simulink model "RB_dyn"  (R2024b)
settings: Solver=ode15s  StartTime=0.0  StopTime=50  RelTol=1e-4
model workspace (MAT data in the model file):
  op_trim1 = opcond.OperatingReport
  op_trim1.Outputs_(1) = opcond.OutputReport
  op_trim1.Outputs_(1).yspec_ = [-24; 8; 2.5]
  op_trim1.Outputs_(1).Block_ = 'RB_dyn/p'
  op_trim1.Outputs_(1).PortWidth_ = 3
  op_trim1.Outputs_(1).PortNumber_ = NaN
  op_trim1.Outputs_(1).y_ = [-24; 8; 2.5]
  op_trim1.Outputs_(1).Known_ = [1; 1; 1]
  op_trim1.Outputs_(1).Min_ = [-Inf; -Inf; -Inf]
  op_trim1.Outputs_(1).Max_ = [Inf; Inf; Inf]
  op_trim1.Outputs_(2) = opcond.OutputReport
  op_trim1.Outputs_(2).yspec_ = [0; 0; 0]
  op_trim1.Outputs_(2).Block_ = 'RB_dyn/omegab'
  op_trim1.Outputs_(2).PortWidth_ = 3
  op_trim1.Outputs_(2).PortNumber_ = NaN
  op_trim1.Outputs_(2).y_ = [-8.63352503319e-27; -2.14269415774e-27; 1.34149458456e-20]
  op_trim1.Outputs_(2).Known_ = [1; 1; 1]
  op_trim1.Outputs_(2).Min_ = [-Inf; -Inf; -Inf]
  op_trim1.Outputs_(2).Max_ = [Inf; Inf; Inf]
  op_trim1.Outputs_(3) = opcond.OutputReport
  op_trim1.Outputs_(3).yspec_ = [0; 0; 0]
  op_trim1.Outputs_(3).Block_ = 'RB_dyn/vi'
  op_trim1.Outputs_(3).PortWidth_ = 3
  op_trim1.Outputs_(3).PortNumber_ = NaN
  op_trim1.Outputs_(3).y_ = [7.32540041679e-34; -1.52127439379e-25; 1.31102361397e-33]
  op_trim1.Outputs_(3).Known_ = [1; 1; 1]
  op_trim1.Outputs_(3).Min_ = [-Inf; -Inf; -Inf]
  op_trim1.Outputs_(3).Max_ = [Inf; Inf; Inf]
  op_trim1.TerminationString_ = 'Operating point specifications were successfully met.'
  op_trim1.OptimizationOutput_.iterations = 4
  op_trim1.OptimizationOutput_.funcCount = 239
  op_trim1.OptimizationOutput_.lssteplength = 1
  op_trim1.OptimizationOutput_.stepsize = 3.80768589581e-07
  op_trim1.OptimizationOutput_.algorithm = 'active-set'
  op_trim1.OptimizationOutput_.firstorderopt = 9.8532065057e-08
  op_trim1.OptimizationOutput_.constrviolation = 2.27373675443e-12
  op_trim1.OptimizationOutput_.message = 'Local minimum found that satisfies the constraints.
    | 
    | Optimization completed because the objective function is non-decreasing in 
    | feasible directions, to within the value of the optimality tolerance,
    | and constraints are satisfied to within the  value of the constraint tolerance.
    | 
    | <stopping criteria details>
    | 
    | Optimization completed: The first-order optimality measure, 9.853207e-08, is less
    | than options.OptimalityTolerance = 1.000000e-06, and the maximum constraint violation,
    | 2.273737e-12,is less than options.ConstraintTolerance = 1.000000e-06.'
  op_trim1.OptimizationOutput_.bestfeasible.x = [-24; 8; 2.5; 7.32541006447e-34; -1.52127439379e-25; 1.31102361397e-33; -8.63352503319e-27; -2.14269415774e-27; 1.34149458456e-20; -24; 8; 2.5; 0; 0; 0; 6.31083339926e-17; -5.82171326753e-17; -2.42996855559e-17; -24; 8; 2.5; 819.705927891; 819.705927891; 819.705927891; 819.705927891; 819.705927891; 819.705927891; 1; -8.92792590779e-26; -9.51340523856e-35; -3.17091829691e-15; 1.43331025767e-22; 2.36799124887e-23; 8.1108698105e-17; 2.21906845952e-21; 7.27462149541e-20; 6.27728709548e-07; -1.96022275097e-15; -1.76674281195e-15; 14.715009237; -0.145; -0.145; 0; 1.39344397348e-34; -1.01153845335e-28; 6.97540031689e-29]
  op_trim1.OptimizationOutput_.bestfeasible.fval = 0
  op_trim1.OptimizationOutput_.bestfeasible.constrviolation = 2.27373675443e-12
  op_trim1.OptimizationOutput_.bestfeasible.firstorderopt = 9.8532065057e-08
  op_trim1.OptimizationOutput_.progress = {'<font face="monospaced"; size=3><BR>', 'Optimizing to solve for all desired dx/dt=0, x(k+1)-x(k)=0, and y=ydes.<BR>', ' <BR>', '(Maximum Error)  Block<BR>', ' ---------------------------------------------------------<BR>', '(1.73412e+03) RB_dyn/Allocation + Actuator Dynamics/Actuator Dynamics/Dinámica Propeller/Integrator<BR>', '(9.66614e-01) RB_dyn/Allocation + Actuator Dynamics/Actuator Dynamics/Dinámica Propeller/Integrator<BR>', '(9.52878e-01) RB_dyn/Allocation + Actuator Dynamics/Actuator Dynamics/Dinámica Propeller/Integrator<BR>', '(1.47056e-04) RB_dyn/Allocation + Actuator Dynamics/Actuator Dynamics/Dinámica Propeller/Integrator<BR>', '(2.27374e-12) RB_dyn/Allocation + Actuator Dynamics/Actuator Dynamics/Dinámica Propeller/Integrator<BR>', '(2.27374e-12) RB_dyn/Allocation + Actuator Dynamics/Actuator Dynamics/Dinámica Propeller/Integrator<BR>', ' <BR>', 'Operating point specifications were successfully met.<BR>'}
  op_trim1.Model_ = 'RB_dyn'
  op_trim1.States_(1) = opcond.StateReport
  op_trim1.States_(1).dx_ = [0; 2.27373675443e-12; 0; 0; 0; 2.27373675443e-12]
  op_trim1.States_(1).Nx_ = 6
  op_trim1.States_(1).Block_ = 'RB_dyn/Allocation + Actuator Dynamics/Actuator Dynamics/Dinámica Propeller/Integrator'
  op_trim1.States_(1).x_ = [819.705927891; 819.705927891; 819.705927891; 819.705927891; 819.705927891; 819.705927891]
  op_trim1.States_(1).SteadyState_ = [1; 1; 1; 1; 1; 1]
  op_trim1.States_(1).dxMin_ = [-Inf; -Inf; -Inf; -Inf; -Inf; -Inf]
  op_trim1.States_(1).dxMax_ = [Inf; Inf; Inf; Inf; Inf; Inf]
  op_trim1.States_(1).Known_ = [0; 0; 0; 0; 0; 0]
  op_trim1.States_(1).Min_ = [-Inf; -Inf; -Inf; -Inf; -Inf; -Inf]
  op_trim1.States_(1).Max_ = [Inf; Inf; Inf; Inf; Inf; Inf]
  op_trim1.States_(2) = opcond.StateReport
  op_trim1.States_(2).dx_ = [7.32540041679e-34; -1.52127439379e-25; 1.31102361397e-33]
  op_trim1.States_(2).Nx_ = 3
  op_trim1.States_(2).Block_ = 'RB_dyn/Dinámica UAV/Rigid Body 
    | dynamics&kinematics
    | /Velocity Integrator'
  op_trim1.States_(2).x_ = [-24; 8; 2.5]
  op_trim1.States_(2).SteadyState_ = [1; 1; 1]
  op_trim1.States_(2).dxMin_ = [-Inf; -Inf; -Inf]
  op_trim1.States_(2).dxMax_ = [Inf; Inf; Inf]
  op_trim1.States_(2).Known_ = [0; 0; 0]
  op_trim1.States_(2).Min_ = [-Inf; -Inf; -Inf]
  op_trim1.States_(2).Max_ = [Inf; Inf; Inf]
  op_trim1.States_(3) = opcond.StateReport
  op_trim1.States_(3).dx_ = [-1.86653566218e-33; 1.75165906311e-24; -1.18423789293e-15; -1.6653345369e-14; 1.11022302464e-14; 3.08218654498e-15]
  op_trim1.States_(3).Nx_ = 6
  op_trim1.States_(3).Block_ = 'RB_dyn/Dinámica UAV/Rigid Body 
    | dynamics&kinematics
    | /nu_b Integrator'
  op_trim1.States_(3).x_ = [7.32541006447e-34; -1.52127439379e-25; 1.31102361397e-33; -8.63352503319e-27; -2.14269415774e-27; 1.34149458456e-20]
  op_trim1.States_(3).SteadyState_ = [1; 1; 1; 1; 1; 1]
  op_trim1.States_(3).dxMin_ = [-Inf; -Inf; -Inf; -Inf; -Inf; -Inf]
  op_trim1.States_(3).dxMax_ = [Inf; Inf; Inf; Inf; Inf; Inf]
  op_trim1.States_(3).Known_ = [0; 0; 0; 0; 0; 0]
  op_trim1.States_(3).Min_ = [-Inf; -Inf; -Inf; -Inf; -Inf; -Inf]
  op_trim1.States_(3).Max_ = [Inf; Inf; Inf; Inf; Inf; Inf]
  op_trim1.States_(4) = opcond.StateReport
  op_trim1.States_(4).dx_ = [2.12688486169e-35; -4.31676251659e-27; -1.07134707887e-27; 6.7074729228e-21]
  op_trim1.States_(4).Nx_ = 4
  op_trim1.States_(4).Block_ = 'RB_dyn/Dinámica UAV/Rigid Body 
    | dynamics&kinematics
    | /q Integrator'
  op_trim1.States_(4).x_ = [1; -8.92792590779e-26; -9.51340523856e-35; -3.17091829691e-15]
  op_trim1.States_(4).SteadyState_ = [1; 1; 1; 1]
  op_trim1.States_(4).dxMin_ = [-Inf; -Inf; -Inf; -Inf]
  op_trim1.States_(4).dxMax_ = [Inf; Inf; Inf; Inf]
  op_trim1.States_(4).Known_ = [0; 0; 0; 0]
  op_trim1.States_(4).Min_ = [-Inf; -Inf; -Inf; -Inf]
  op_trim1.States_(4).Max_ = [Inf; Inf; Inf; Inf]
  op_trim1.States_(5) = opcond.StateReport
  op_trim1.States_(5).dx_ = [-7.32540041679e-34; 1.52127439379e-25; -1.31102361397e-33]
  op_trim1.States_(5).Nx_ = 3
  op_trim1.States_(5).Block_ = 'RB_dyn/Position Controller/ Bl Controller/ev integrator'
  op_trim1.States_(5).x_ = [1.43331025767e-22; 2.36799124887e-23; 8.1108698105e-17]
  op_trim1.States_(5).SteadyState_ = [1; 1; 1]
  op_trim1.States_(5).dxMin_ = [-Inf; -Inf; -Inf]
  op_trim1.States_(5).dxMax_ = [Inf; Inf; Inf]
  op_trim1.States_(5).Known_ = [0; 0; 0]
  op_trim1.States_(5).Min_ = [-Inf; -Inf; -Inf]
  op_trim1.States_(5).Max_ = [Inf; Inf; Inf]
  op_trim1.States_(6) = opcond.StateReport
  op_trim1.States_(6).dx_ = 1.1863912976e-33
  op_trim1.States_(6).Nx_ = 1
  op_trim1.States_(6).Block_ = 'RB_dyn/Predictor/Adaptive Laws/Projection and integration /Projection Cx/Integrator'
  op_trim1.States_(6).x_ = -1.96022275097e-15
  op_trim1.States_(6).SteadyState_ = 1
  op_trim1.States_(6).dxMin_ = -Inf
  op_trim1.States_(6).dxMax_ = Inf
  op_trim1.States_(6).Known_ = 0
  op_trim1.States_(6).Min_ = -Inf
  op_trim1.States_(6).Max_ = Inf
  op_trim1.States_(7) = opcond.StateReport
  op_trim1.States_(7).dx_ = -3.04052571068e-25
  op_trim1.States_(7).Nx_ = 1
  op_trim1.States_(7).Block_ = 'RB_dyn/Predictor/Adaptive Laws/Projection and integration /Projection Cy/Integrator'
  op_trim1.States_(7).x_ = -1.76674281195e-15
  op_trim1.States_(7).SteadyState_ = 1
  op_trim1.States_(7).dxMin_ = -Inf
  op_trim1.States_(7).dxMax_ = Inf
  op_trim1.States_(7).Known_ = 0
  op_trim1.States_(7).Min_ = -Inf
  op_trim1.States_(7).Max_ = Inf
  op_trim1.States_(8) = opcond.StateReport
  op_trim1.States_(8).dx_ = 4.65017947635e-29
  op_trim1.States_(8).Nx_ = 1
  op_trim1.States_(8).Block_ = 'RB_dyn/Predictor/Adaptive Laws/Projection and integration /Projection Cz/Integrator'
  op_trim1.States_(8).x_ = 14.715009237
  op_trim1.States_(8).SteadyState_ = 1
  op_trim1.States_(8).dxMin_ = -Inf
  op_trim1.States_(8).dxMax_ = Inf
  op_trim1.States_(8).Known_ = 0
  op_trim1.States_(8).Min_ = -Inf
  op_trim1.States_(8).Max_ = Inf
  op_trim1.States_(9) = opcond.StateReport
  op_trim1.States_(9).dx_ = 1.0489814806e-27
  op_trim1.States_(9).Nx_ = 1
  op_trim1.States_(9).Block_ = 'RB_dyn/Predictor/Adaptive Laws/Projection and integration /Projection Dx/Integrator'
  op_trim1.States_(9).x_ = -0.145
  op_trim1.States_(9).SteadyState_ = 1
  op_trim1.States_(9).dxMin_ = -Inf
  op_trim1.States_(9).dxMax_ = Inf
  op_trim1.States_(9).Known_ = 0
  op_trim1.States_(9).Min_ = -Inf
  op_trim1.States_(9).Max_ = Inf
  op_trim1.States_(10) = opcond.StateReport
  op_trim1.States_(10).dx_ = 1.0489814806e-27
  op_trim1.States_(10).Nx_ = 1
  op_trim1.States_(10).Block_ = 'RB_dyn/Predictor/Adaptive Laws/Projection and integration /Projection Dy/Integrator'
  op_trim1.States_(10).x_ = -0.145
  op_trim1.States_(10).SteadyState_ = 1
  op_trim1.States_(10).dxMin_ = -Inf
  op_trim1.States_(10).dxMax_ = Inf
  op_trim1.States_(10).Known_ = 0
  op_trim1.States_(10).Min_ = -Inf
  op_trim1.States_(10).Max_ = Inf
  op_trim1.States_(11) = opcond.StateReport
  op_trim1.States_(11).dx_ = 6.68915726758e-29
  op_trim1.States_(11).Nx_ = 1
  op_trim1.States_(11).Block_ = 'RB_dyn/Predictor/Adaptive Laws/Projection and integration /Projection Dz/Integrator'
  op_trim1.States_(11).SteadyState_ = 1
  op_trim1.States_(11).dxMin_ = -Inf
  op_trim1.States_(11).dxMax_ = Inf
  op_trim1.States_(11).Known_ = 0
  op_trim1.States_(11).Min_ = -Inf
  op_trim1.States_(11).Max_ = Inf
  op_trim1.States_(12) = opcond.StateReport
  op_trim1.States_(12).dx_ = 4.56078904608e-28
  op_trim1.States_(12).Nx_ = 1
  op_trim1.States_(12).Block_ = 'RB_dyn/Predictor/Adaptive Laws/Projection and integration /Projection lambda1/Integrator'
  op_trim1.States_(12).x_ = 2.21906845952e-21
  op_trim1.States_(12).SteadyState_ = 1
  op_trim1.States_(12).dxMin_ = -Inf
  op_trim1.States_(12).dxMax_ = Inf
  op_trim1.States_(12).Known_ = 0
  op_trim1.States_(12).Min_ = -Inf
  op_trim1.States_(12).Max_ = Inf
  op_trim1.States_(13) = opcond.StateReport
  op_trim1.States_(13).dx_ = 4.56078904608e-28
  op_trim1.States_(13).Nx_ = 1
  op_trim1.States_(13).Block_ = 'RB_dyn/Predictor/Adaptive Laws/Projection and integration /Projection lambda2/Integrator'
  op_trim1.States_(13).x_ = 7.27462149541e-20
  op_trim1.States_(13).SteadyState_ = 1
  op_trim1.States_(13).dxMin_ = -Inf
  op_trim1.States_(13).dxMax_ = Inf
  op_trim1.States_(13).Known_ = 0
  op_trim1.States_(13).Min_ = -Inf
  op_trim1.States_(13).Max_ = Inf
  op_trim1.States_(14) = opcond.StateReport
  op_trim1.States_(14).dx_ = 2.5079644533e-28
  op_trim1.States_(14).Nx_ = 1
  op_trim1.States_(14).Block_ = 'RB_dyn/Predictor/Adaptive Laws/Projection and integration /Projection lambda3/Integrator'
  op_trim1.States_(14).x_ = 6.27728709548e-07
  op_trim1.States_(14).SteadyState_ = 1
  op_trim1.States_(14).dxMin_ = -Inf
  op_trim1.States_(14).dxMax_ = Inf
  op_trim1.States_(14).Known_ = 0
  op_trim1.States_(14).Min_ = -Inf
  op_trim1.States_(14).Max_ = Inf
  op_trim1.States_(15) = opcond.StateReport
  op_trim1.States_(15).dx_ = [9.55540155376e-24; -1.12718460583e-24; -1.3950538429e-27]
  op_trim1.States_(15).Nx_ = 3
  op_trim1.States_(15).Block_ = 'RB_dyn/Predictor/Predictor Dynamics/v_hat_int'
  op_trim1.States_(15).x_ = [1.39344397348e-34; -1.01153845335e-28; 6.97540031689e-29]
  op_trim1.States_(15).SteadyState_ = [1; 1; 1]
  op_trim1.States_(15).dxMin_ = [-Inf; -Inf; -Inf]
  op_trim1.States_(15).dxMax_ = [Inf; Inf; Inf]
  op_trim1.States_(15).Known_ = [0; 0; 0]
  op_trim1.States_(15).Min_ = [-Inf; -Inf; -Inf]
  op_trim1.States_(15).Max_ = [Inf; Inf; Inf]
  op_trim1.States_(16) = opcond.StateReport
  op_trim1.States_(16).dx_ = [0; 0; 0; 0; 0; 0; 0; 0; 0]
  op_trim1.States_(16).Nx_ = 9
  op_trim1.States_(16).Block_ = 'RB_dyn/Ref State Space/Integrator'
  op_trim1.States_(16).x_ = [-24; 8; 2.5; 0; 0; 0; 6.31083339926e-17; -5.82171326753e-17; -2.42996855559e-17]
  op_trim1.States_(16).SteadyState_ = [1; 1; 1; 1; 1; 1; 1; 1; 1]
  op_trim1.States_(16).dxMin_ = [-Inf; -Inf; -Inf; -Inf; -Inf; -Inf; -Inf; -Inf; -Inf]
  op_trim1.States_(16).dxMax_ = [Inf; Inf; Inf; Inf; Inf; Inf; Inf; Inf; Inf]
  op_trim1.States_(16).Known_ = [0; 0; 0; 0; 0; 0; 0; 0; 0]
  op_trim1.States_(16).Min_ = [-Inf; -Inf; -Inf; -Inf; -Inf; -Inf; -Inf; -Inf; -Inf]
  op_trim1.States_(16).Max_ = [Inf; Inf; Inf; Inf; Inf; Inf; Inf; Inf; Inf]
  op_trim1.States_(17) = opcond.StateReport
  op_trim1.States_(17).dx_ = [0; 0; 0]
  op_trim1.States_(17).Nx_ = 3
  op_trim1.States_(17).Block_ = 'RB_dyn/V limitation/v_cmd integrator'
  op_trim1.States_(17).x_ = [-24; 8; 2.5]
  op_trim1.States_(17).SteadyState_ = [1; 1; 1]
  op_trim1.States_(17).dxMin_ = [-Inf; -Inf; -Inf]
  op_trim1.States_(17).dxMax_ = [Inf; Inf; Inf]
  op_trim1.States_(17).Known_ = [0; 0; 0]
  op_trim1.States_(17).Min_ = [-Inf; -Inf; -Inf]
  op_trim1.States_(17).Max_ = [Inf; Inf; Inf]
  op_trim2 = opcond.OperatingReport
  op_trim2.Outputs_(1) = opcond.OutputReport
  op_trim2.Outputs_(1).yspec_ = [0; 0; 0]
  op_trim2.Outputs_(1).Block_ = 'RB_dyn/p'
  op_trim2.Outputs_(1).PortWidth_ = 3
  op_trim2.Outputs_(1).PortNumber_ = NaN
  op_trim2.Outputs_(1).y_ = [0.00247480136454; 1.78220997909e-05; 1.00066556681]
  op_trim2.Outputs_(1).Known_ = [0; 0; 0]
  op_trim2.Outputs_(1).Min_ = [-Inf; -Inf; -Inf]
  op_trim2.Outputs_(1).Max_ = [Inf; Inf; Inf]
  op_trim2.Outputs_(2) = opcond.OutputReport
  op_trim2.Outputs_(2).yspec_ = [0; 0; 0]
  op_trim2.Outputs_(2).Block_ = 'RB_dyn/omegab'
  op_trim2.Outputs_(2).PortWidth_ = 3
  op_trim2.Outputs_(2).PortNumber_ = NaN
  op_trim2.Outputs_(2).y_ = [3.33045179926e-22; 5.43985403482e-20; 1.33504882827e-20]
  op_trim2.Outputs_(2).Known_ = [1; 1; 1]
  op_trim2.Outputs_(2).Min_ = [-Inf; -Inf; -Inf]
  op_trim2.Outputs_(2).Max_ = [Inf; Inf; Inf]
  op_trim2.Outputs_(3) = opcond.OutputReport
  op_trim2.Outputs_(3).yspec_ = [2; 0; 0]
  op_trim2.Outputs_(3).Block_ = 'RB_dyn/vb'
  op_trim2.Outputs_(3).PortWidth_ = 3
  op_trim2.Outputs_(3).PortNumber_ = NaN
  op_trim2.Outputs_(3).y_ = [2; 4.03619005258e-20; 4.67904532738e-20]
  op_trim2.Outputs_(3).Known_ = [1; 1; 1]
  op_trim2.Outputs_(3).Min_ = [-Inf; -Inf; -Inf]
  op_trim2.Outputs_(3).Max_ = [Inf; Inf; Inf]
  op_trim2.Outputs_(4) = opcond.OutputReport
  op_trim2.Outputs_(4).yspec_ = [0; 0; 0; 0]
  op_trim2.Outputs_(4).Block_ = 'RB_dyn/q_dot'
  op_trim2.Outputs_(4).PortWidth_ = 4
  op_trim2.Outputs_(4).PortNumber_ = NaN
  op_trim2.Outputs_(4).y_ = [-1.22708523425e-22; 2.15491260397e-22; 2.71988790305e-20; 6.67430878408e-21]
  op_trim2.Outputs_(4).Known_ = [1; 1; 1; 1]
  op_trim2.Outputs_(4).Min_ = [-Inf; -Inf; -Inf; -Inf]
  op_trim2.Outputs_(4).Max_ = [Inf; Inf; Inf; Inf]
  op_trim2.TerminationString_ = 'Operating point specifications were successfully met.'
  op_trim2.OptimizationOutput_.iterations = 4
  op_trim2.OptimizationOutput_.funcCount = 83
  op_trim2.OptimizationOutput_.lssteplength = 1
  op_trim2.OptimizationOutput_.stepsize = 0.000853707830083
  op_trim2.OptimizationOutput_.algorithm = 'active-set'
  op_trim2.OptimizationOutput_.firstorderopt = 0
  op_trim2.OptimizationOutput_.constrviolation = 4.86637581906e-09
  op_trim2.OptimizationOutput_.message = 'Local minimum found that satisfies the constraints.
    | 
    | Optimization completed because the objective function is non-decreasing in 
    | feasible directions, to within the value of the optimality tolerance,
    | and constraints are satisfied to within the  value of the constraint tolerance.
    | 
    | <stopping criteria details>
    | 
    | Optimization completed: The first-order optimality measure, 0.000000e+00, is less
    | than options.OptimalityTolerance = 1.000000e-06, and the maximum constraint violation,
    | 4.866376e-09,is less than options.ConstraintTolerance = 1.000000e-06.'
  op_trim2.OptimizationOutput_.bestfeasible.x = [0.00247480136454; 1.78220997909e-05; 1.00066556681; 2; 4.03619005258e-20; 4.67904532738e-20; 3.33045179926e-22; 5.43985403482e-20; 1.33504882827e-20; 1.00130830579; -3.05904618209e-06; 0.00467811367405; -0.000654708249021; 733.164421503; 733.163541763; 733.164247408; 733.164421503; 733.163541763; 733.164247408]
  op_trim2.OptimizationOutput_.bestfeasible.fval = 0
  op_trim2.OptimizationOutput_.bestfeasible.constrviolation = 4.86637581906e-09
  op_trim2.OptimizationOutput_.bestfeasible.firstorderopt = 0
  op_trim2.OptimizationOutput_.progress = {'<font face="monospaced"; size=3><BR>', 'Optimizing to solve for all desired dx/dt=0, x(k+1)-x(k)=0, and y=ydes.<BR>', ' <BR>', '(Maximum Error)  Block<BR>', ' ---------------------------------------------------------<BR>', '(2.00000e+00) RB_dyn/vb<BR>', '(3.56041e-04) RB_dyn/Dinámica UAV/Rigid Body  dynamics&kinematics /Integrator1<BR>', '(2.35344e-06) RB_dyn/Dinámica UAV/Rigid Body  dynamics&kinematics /Integrator1<BR>', '(4.86638e-09) RB_dyn/Dinámica UAV/Rigid Body  dynamics&kinematics /Integrator1<BR>', '(4.86638e-09) RB_dyn/Dinámica UAV/Rigid Body  dynamics&kinematics /Integrator1<BR>', ' <BR>', 'Operating point specifications were successfully met.<BR>'}
  op_trim2.Model_ = 'RB_dyn'
  op_trim2.States_(1) = opcond.StateReport
  op_trim2.States_(1).dx_ = [1.9999109815; -0.00261541012492; -0.0186875811863]
  op_trim2.States_(1).Nx_ = 3
  op_trim2.States_(1).Block_ = 'RB_dyn/Dinámica UAV/Rigid Body 
    | dynamics&kinematics
    | /Integrator'
  op_trim2.States_(1).x_ = [0.00247480136454; 1.78220997909e-05; 1.00066556681]
  op_trim2.States_(1).SteadyState_ = [0; 0; 0]
  op_trim2.States_(1).dxMin_ = [-Inf; -Inf; -Inf]
  op_trim2.States_(1).dxMax_ = [Inf; Inf; Inf]
  op_trim2.States_(1).Known_ = [0; 0; 0]
  op_trim2.States_(1).Min_ = [-Inf; -Inf; -Inf]
  op_trim2.States_(1).Max_ = [Inf; Inf; Inf]
  op_trim2.States_(2) = opcond.StateReport
  op_trim2.States_(2).dx_ = [-9.33392610888e-10; 4.86637581906e-09; 2.34032053105e-10; 9.99200562301e-14; 2.22041993795e-13; 2.31278885321e-14]
  op_trim2.States_(2).Nx_ = 6
  op_trim2.States_(2).Block_ = 'RB_dyn/Dinámica UAV/Rigid Body 
    | dynamics&kinematics
    | /Integrator1'
  op_trim2.States_(2).x_ = [2; 4.03619005258e-20; 4.67904532738e-20; 3.33045179926e-22; 5.43985403482e-20; 1.33504882827e-20]
  op_trim2.States_(2).SteadyState_ = [1; 1; 1; 1; 1; 1]
  op_trim2.States_(2).dxMin_ = [-Inf; -Inf; -Inf; -Inf; -Inf; -Inf]
  op_trim2.States_(2).dxMax_ = [Inf; Inf; Inf; Inf; Inf; Inf]
  op_trim2.States_(2).Known_ = [0; 0; 0; 0; 0; 0]
  op_trim2.States_(2).Min_ = [-Inf; -Inf; -Inf; -Inf; -Inf; -Inf]
  op_trim2.States_(2).Max_ = [Inf; Inf; Inf; Inf; Inf; Inf]
  op_trim2.States_(3) = opcond.StateReport
  op_trim2.States_(3).dx_ = [-1.22708523425e-22; 2.15491260397e-22; 2.71988790305e-20; 6.67430878408e-21]
  op_trim2.States_(3).Nx_ = 4
  op_trim2.States_(3).Block_ = 'RB_dyn/Dinámica UAV/Rigid Body 
    | dynamics&kinematics
    | /Integrator2'
  op_trim2.States_(3).x_ = [1.00130830579; -3.05904618209e-06; 0.00467811367405; -0.000654708249021]
  op_trim2.States_(3).SteadyState_ = [1; 1; 1; 1]
  op_trim2.States_(3).dxMin_ = [-Inf; -Inf; -Inf; -Inf]
  op_trim2.States_(3).dxMax_ = [Inf; Inf; Inf; Inf]
  op_trim2.States_(3).Known_ = [0; 0; 0; 0]
  op_trim2.States_(3).Min_ = [-Inf; -Inf; -Inf; -Inf]
  op_trim2.States_(3).Max_ = [Inf; Inf; Inf; Inf]
  op_trim2.Inputs_ = opcond.InputReport
  op_trim2.Inputs_.Block_ = 'RB_dyn/w_c1'
  op_trim2.Inputs_.PortWidth_ = 6
  op_trim2.Inputs_.PortDimensions_ = [2 6 1]
  op_trim2.Inputs_.u_ = [733.164421503; 733.163541763; 733.164247408; 733.164421503; 733.163541763; 733.164247408]
  op_trim2.Inputs_.Known_ = [0; 0; 0; 0; 0; 0]
  op_trim2.Inputs_.Min_ = [-Inf; -Inf; -Inf; -Inf; -Inf; -Inf]
  op_trim2.Inputs_.Max_ = [Inf; Inf; Inf; Inf; Inf; Inf]
  op_trim3 = opcond.OperatingReport
  op_trim3.Outputs_(1) = opcond.OutputReport
  op_trim3.Outputs_(1).yspec_ = [0; 0; 1]
  op_trim3.Outputs_(1).Block_ = 'RB_dyn/p'
  op_trim3.Outputs_(1).PortWidth_ = 3
  op_trim3.Outputs_(1).PortNumber_ = NaN
  op_trim3.Outputs_(1).y_ = [2; 1.8997500259e-19; 1]
  op_trim3.Outputs_(1).Known_ = [0; 1; 1]
  op_trim3.Outputs_(1).Min_ = [-Inf; -Inf; -Inf]
  op_trim3.Outputs_(1).Max_ = [Inf; Inf; Inf]
  op_trim3.Outputs_(2) = opcond.OutputReport
  op_trim3.Outputs_(2).yspec_ = [0; 0; 0]
  op_trim3.Outputs_(2).Block_ = 'RB_dyn/omegab'
  op_trim3.Outputs_(2).PortWidth_ = 3
  op_trim3.Outputs_(2).PortNumber_ = NaN
  op_trim3.Outputs_(2).y_ = [4.96522925532e-21; -1.00432731025e-20; 2.86594702329e-22]
  op_trim3.Outputs_(2).Known_ = [1; 1; 1]
  op_trim3.Outputs_(2).Min_ = [-Inf; -Inf; -Inf]
  op_trim3.Outputs_(2).Max_ = [Inf; Inf; Inf]
  op_trim3.Outputs_(3) = opcond.OutputReport
  op_trim3.Outputs_(3).yspec_ = [2; 0; 0]
  op_trim3.Outputs_(3).Block_ = 'RB_dyn/vi'
  op_trim3.Outputs_(3).PortWidth_ = 3
  op_trim3.Outputs_(3).PortNumber_ = NaN
  op_trim3.Outputs_(3).y_ = [1.99999999584; 3.36919514236e-13; 2.51599609202e-11]
  op_trim3.Outputs_(3).Known_ = [1; 1; 1]
  op_trim3.Outputs_(3).Min_ = [-Inf; -Inf; -Inf]
  op_trim3.Outputs_(3).Max_ = [Inf; Inf; Inf]
  op_trim3.Outputs_(4) = opcond.OutputReport
  op_trim3.Outputs_(4).yspec_ = [0; 0; 0; 0]
  op_trim3.Outputs_(4).Block_ = 'RB_dyn/q_dot'
  op_trim3.Outputs_(4).PortWidth_ = 4
  op_trim3.Outputs_(4).PortNumber_ = NaN
  op_trim3.Outputs_(4).y_ = [2.34608367838e-23; 2.48325700153e-21; -5.02158175194e-21; 1.31697135121e-22]
  op_trim3.Outputs_(4).Known_ = [1; 1; 1; 1]
  op_trim3.Outputs_(4).Min_ = [-Inf; -Inf; -Inf; -Inf]
  op_trim3.Outputs_(4).Max_ = [Inf; Inf; Inf; Inf]
  op_trim3.TerminationString_ = 'Operating point specifications were successfully met.'
  op_trim3.OptimizationOutput_.iterations = 3
  op_trim3.OptimizationOutput_.funcCount = 62
  op_trim3.OptimizationOutput_.lssteplength = 1
  op_trim3.OptimizationOutput_.stepsize = 2.51866712373e-07
  op_trim3.OptimizationOutput_.algorithm = 'active-set'
  op_trim3.OptimizationOutput_.firstorderopt = 0
  op_trim3.OptimizationOutput_.constrviolation = 4.16122736269e-09
  op_trim3.OptimizationOutput_.message = 'Local minimum found that satisfies the constraints.
    | 
    | Optimization completed because the objective function is non-decreasing in 
    | feasible directions, to within the value of the optimality tolerance,
    | and constraints are satisfied to within the  value of the constraint tolerance.
    | 
    | <stopping criteria details>
    | 
    | Optimization completed: The first-order optimality measure, 0.000000e+00, is less
    | than options.OptimalityTolerance = 1.000000e-06, and the maximum constraint violation,
    | 4.161227e-09,is less than options.ConstraintTolerance = 1.000000e-06.'
  op_trim3.OptimizationOutput_.bestfeasible.x = [2; 1.8997500259e-19; 1; 1.99991268736; 7.90764284672e-09; 0.0186875973027; 4.96522925532e-21; -1.00432731025e-20; 2.86594702329e-22; 0.990003847282; -9.14762811649e-12; 0.0046252992669; -1.95715128224e-09; 733.164070314; 733.164070327; 733.164070314; 733.164070314; 733.164070327; 733.164070314]
  op_trim3.OptimizationOutput_.bestfeasible.fval = 0
  op_trim3.OptimizationOutput_.bestfeasible.constrviolation = 4.16122736269e-09
  op_trim3.OptimizationOutput_.bestfeasible.firstorderopt = 0
  op_trim3.OptimizationOutput_.progress = {'<font face="monospaced"; size=3><BR>', 'Optimizing to solve for all desired dx/dt=0, x(k+1)-x(k)=0, and y=ydes.<BR>', ' <BR>', '(Maximum Error)  Block<BR>', ' ---------------------------------------------------------<BR>', '(2.00000e+00) RB_dyn/vi<BR>', '(2.27281e-02) RB_dyn/vi<BR>', '(4.16123e-09) RB_dyn/vi<BR>', '(4.16123e-09) RB_dyn/vi<BR>', ' <BR>', 'Operating point specifications were successfully met.<BR>'}
  op_trim3.Model_ = 'RB_dyn'
  op_trim3.States_(1) = opcond.StateReport
  op_trim3.States_(1).dx_ = [1.99999999584; 3.36919514236e-13; 2.51599609202e-11]
  op_trim3.States_(1).Nx_ = 3
  op_trim3.States_(1).Block_ = 'RB_dyn/Dinámica UAV/Rigid Body 
    | dynamics&kinematics
    | /Velocity Integrator'
  op_trim3.States_(1).x_ = [2; 1.8997500259e-19; 1]
  op_trim3.States_(1).SteadyState_ = [0; 1; 0]
  op_trim3.States_(1).dxMin_ = [-Inf; -Inf; -Inf]
  op_trim3.States_(1).dxMax_ = [Inf; Inf; Inf]
  op_trim3.States_(1).Known_ = [0; 0; 0]
  op_trim3.States_(1).Min_ = [-Inf; -Inf; -Inf]
  op_trim3.States_(1).Max_ = [Inf; Inf; Inf]
  op_trim3.States_(2) = opcond.StateReport
  op_trim3.States_(2).dx_ = [-7.23842280532e-14; 6.0161035039e-14; 2.75043099405e-09; -8.74300655725e-12; -3.87467787386e-12; 1.20890947797e-12]
  op_trim3.States_(2).Nx_ = 6
  op_trim3.States_(2).Block_ = 'RB_dyn/Dinámica UAV/Rigid Body 
    | dynamics&kinematics
    | /nu_b Integrator'
  op_trim3.States_(2).x_ = [1.99991268736; 7.90764284672e-09; 0.0186875973027; 4.96522925532e-21; -1.00432731025e-20; 2.86594702329e-22]
  op_trim3.States_(2).SteadyState_ = [1; 1; 1; 1; 1; 1]
  op_trim3.States_(2).dxMin_ = [-Inf; -Inf; -Inf; -Inf; -Inf; -Inf]
  op_trim3.States_(2).dxMax_ = [Inf; Inf; Inf; Inf; Inf; Inf]
  op_trim3.States_(2).Known_ = [0; 0; 0; 0; 0; 0]
  op_trim3.States_(2).Min_ = [-Inf; -Inf; -Inf; -Inf; -Inf; -Inf]
  op_trim3.States_(2).Max_ = [Inf; Inf; Inf; Inf; Inf; Inf]
  op_trim3.States_(3) = opcond.StateReport
  op_trim3.States_(3).dx_ = [2.34608367838e-23; 2.48325700153e-21; -5.02158175194e-21; 1.31697135121e-22]
  op_trim3.States_(3).Nx_ = 4
  op_trim3.States_(3).Block_ = 'RB_dyn/Dinámica UAV/Rigid Body 
    | dynamics&kinematics
    | /q Integrator'
  op_trim3.States_(3).x_ = [0.990003847282; -9.14762811649e-12; 0.0046252992669; -1.95715128224e-09]
  op_trim3.States_(3).SteadyState_ = [1; 1; 1; 1]
  op_trim3.States_(3).dxMin_ = [-Inf; -Inf; -Inf; -Inf]
  op_trim3.States_(3).dxMax_ = [Inf; Inf; Inf; Inf]
  op_trim3.States_(3).Known_ = [0; 0; 0; 0]
  op_trim3.States_(3).Min_ = [-Inf; -Inf; -Inf; -Inf]
  op_trim3.States_(3).Max_ = [Inf; Inf; Inf; Inf]
  op_trim3.Inputs_ = opcond.InputReport
  op_trim3.Inputs_.Block_ = 'RB_dyn/w_c1'
  op_trim3.Inputs_.PortWidth_ = 6
  op_trim3.Inputs_.PortDimensions_ = [2 6 1]
  op_trim3.Inputs_.u_ = [733.164070314; 733.164070327; 733.164070314; 733.164070314; 733.164070327; 733.164070314]
  op_trim3.Inputs_.Known_ = [0; 0; 0; 0; 0; 0]
  op_trim3.Inputs_.Min_ = [-Inf; -Inf; -Inf; -Inf; -Inf; -Inf]
  op_trim3.Inputs_.Max_ = [Inf; Inf; Inf; Inf; Inf; Inf]
values from neighbouring files (symbols this model uses):
  B_p = 1/(m_t_est)    [MAIN_exam_2025.m]
  F_matrix = zeros(6, 6)    [MAIN_exam_2025.m]
  Finv = pinv(F_matrix)    [MAIN_exam_2025.m]
  GAMMA_a = diag([0.5, 0.5, 0.5,1, 1, 1, 1, 1, 1, 1])    [MAIN_exam_2025.m]
  k_f = 3.65e-6    (= 3.65e-06)    [MAIN_exam_2025.m]
  K_position = diag([K_px, K_py, K_pz])    [MAIN_exam_2025.m]
  Ki = diag([K_ix, K_iy, K_iz])    [MAIN_exam_2025.m]
  Kp = diag([K_dx, K_dy, K_dz])    [MAIN_exam_2025.m]
  L = 100    [MAIN_exam_2025.m]
  LAMBDA_hat_0 = ones(3,1)    [MAIN_exam_2025.m]
  Lambda_matrix = diag([1, 1, 1, 1,1, 1])    [MAIN_exam_2025.m]
  m_t_est = UAV.m0 + m_p    [MAIN_exam_2025.m]
  omegab_0 = [0 0 0]'    [MAIN_exam_2025.m]
  p_0 = [-24 8 2.5]'    [MAIN_exam_2025.m]
  p_x_data = p_lookup(:,1)    [MAIN_exam_2025.m]
  p_y_data = p_lookup(:,2)    [MAIN_exam_2025.m]
  p_z_data = p_lookup(:,3)    [MAIN_exam_2025.m]
  q_0 = eul2quat([0, 0, 0 ]*degToRad,'XYZ')'    [MAIN_exam_2025.m]
  t_lookup = ts_pos.Time    [MAIN_exam_2025.m]
  Theta_0 = [0;0;(m_t_est)*par.g;D_fv_bar(1,1);D_fv_bar(2,2);D_fv_bar(3,3)]    [MAIN_exam_2025.m]
  v_0 = R_0*vb_0    [MAIN_exam_2025.m]
  vb_0 = [0 0 0]'    [MAIN_exam_2025.m]
undefined symbols (not defined in the file or in its folder): ctrl, par, proj, UAV
(part 1 of 2)
settings Model: PacingRate=10  Creator=justs  LastModifiedBy=fjmno
settings DataIOCC: ExternalInput=getinputstruct(op_trim1)  InitialState=getstatestruct(op_trim1)
settings OptimizationCC: ReuseModelBlockBuffer=off
settings ModelReferenceCC: EnableRefExpFcnMdlSchedulingChecks=on
settings RTWCC: GPUComputeCapability=3.5

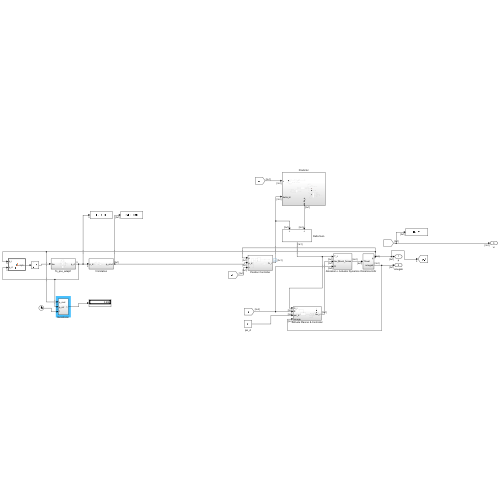
[thumbnail: Simulink's stored preview of the top-level diagram]
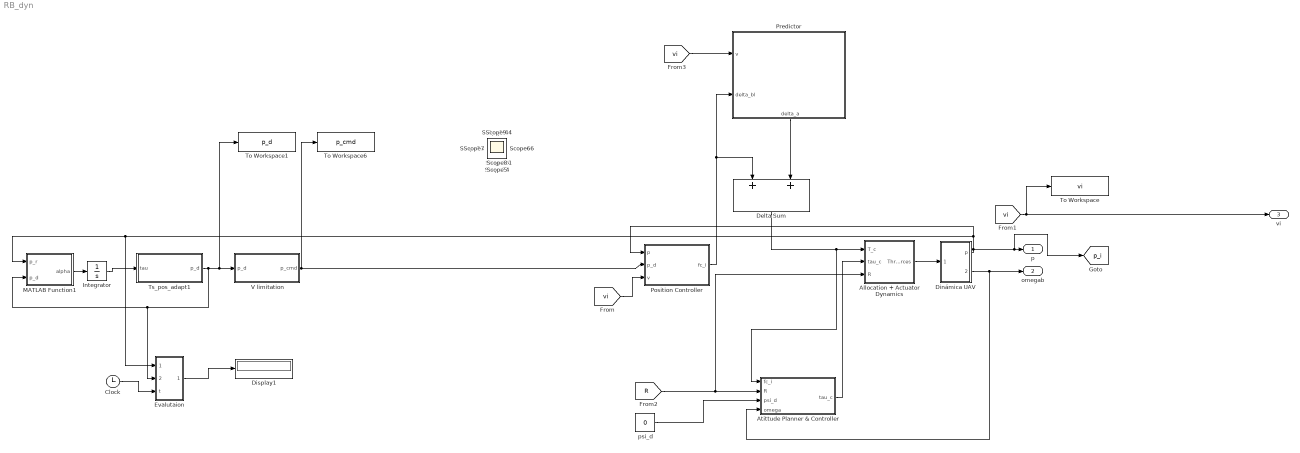
== system RB_dyn ==
  Allocation + Actuator Dynamics : Subsystem
  Atittude Planner & Controller : Subsystem
  Clock : Clock
  Delta Sum : Sum
  Dinámica UAV : Subsystem
  Display1 : Display
  Evalutaion : Subsystem
  Integrator : Integrator  LimitOutput=on  UpperSaturationLimit=100  LowerSaturationLimit=0
  MATLAB Function1 : MATLAB Function  TreatAsAtomicUnit=on
  Position Controller : Subsystem
  Predictor : Subsystem
      settings: PortSchema="{\"entries\":[{\"content\":{\"sides\":[{\"content\":{\"connectorIds\":[\"In1\",\"In2\"]},\"type\":\"ConnectorPlacement.EquallySpacedRectSide\",\"uuid\":\"2d7e5448-a673-4ee6-9554-3ae3da0510a7\"},{\"content\":{\"side\":\"RIGHT\"},\"type\":\"ConnectorPlacement.EquallySpacedRectSide\",\"uuid\":\"bdb394af-b14b-4430-b0f8-1c11ee2cd103\"},{\"content\":{\"side\":\"TOP\"},\"type\":\"ConnectorPlacement.EquallySpacedRectSide\",\"uuid\":\"33e4180b-1495-4b61-9946-a5cb762c2be0\"},{\"content\":{\"connectorIds\":[\"Out1\"],\"side\":\"BOTTOM\"},\"type\":\"ConnectorPlacement.EquallySpacedRectSide\",\"uuid\":\"431cb0aa-f168-4440-940a-a54a9a698ac8\"}]},\"type\":\"ConnectorPlacement.EquallySpacedConnector\",\"uuid\":\"3d6a6a3c-444f-43bb-b75d-620492f88baa\"}],\"packageUris\":[\"http://schema.mathworks.com/mf0/Connector/R2020b\"],\"version\":\"1.0\"}"
  To Workspace : ToWorkspace  VariableName=vi  SaveFormat=Timeseries  SampleTime=-1
  To Workspace1 : ToWorkspace  VariableName=p_d  SaveFormat=Timeseries  SampleTime=-1
  To Workspace6 : ToWorkspace  VariableName=p_cmd  SaveFormat=Timeseries  SampleTime=-1
  Ts_pos_adapt1 : Subsystem
  V limitation : Subsystem
  psi_d : Constant  Value=0
  p : Outport  PortDimensions=[3,1]
  omegab : Outport  Port=2
  vi : Outport  Port=3
  Scope{,1..14,18..21,23..24,26} (22 alike) : Scope
  tag scope: p_i=global
  wires:
  Dinámica UAV/2(omegab) -> Atittude Planner & Controller/4(omega), omegab/1
  Allocation + Actuator Dynamics/1(Thrust_forces) -> Dinámica UAV/1(Thrust)
  [R] -> Allocation + Actuator Dynamics/3(R), Atittude Planner & Controller/2(R)
  Delta Sum/1 -> Atittude Planner & Controller/1(fc_i), Allocation + Actuator Dynamics/1(T_c)
  Position Controller/1(fc_i) -> Delta Sum/1, Predictor/2(delta_bl)
  V limitation/1(p_cmd) -> Position Controller/2(p_d), To Workspace6/1
  [vi] -> Position Controller/3(v)
  [vi] -> Predictor/1(v)
  Atittude Planner & Controller/1(tau_c) -> Allocation + Actuator Dynamics/2(tau_c)
  Dinámica UAV/1(p) -> Position Controller/1(p), Evalutaion/1(p_real), MATLAB Function1/1(p_r), p/1, [p_i]
  psi_d/1 -> Atittude Planner & Controller/3(psi_d)
  MATLAB Function1/1(alpha) -> Integrator/1
  Integrator/1 -> Ts_pos_adapt1/1(tau)
  Ts_pos_adapt1/1(p_d) -> Evalutaion/2(p_ref), MATLAB Function1/2(p_d), To Workspace1/1, V limitation/1(p_d)
  Predictor/1(delta_a) -> Delta Sum/2
  Evalutaion/1(Out1) -> Display1/1
  Clock/1 -> Evalutaion/3(t)
  [vi] -> vi/1, To Workspace/1

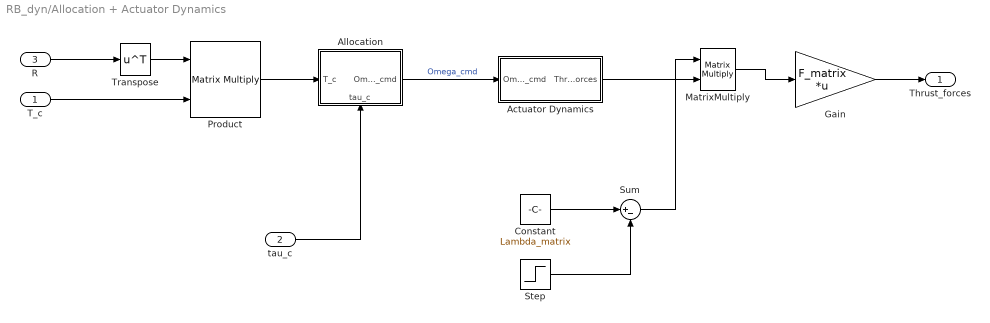
== system RB_dyn/Allocation + Actuator Dynamics ==
  T_c : Inport
  tau_c : Inport  Port=2
  R : Inport  Port=3
  Actuator Dynamics : Subsystem
  Allocation : Subsystem
      settings: PortSchema="{\"entries\":[{\"content\":{\"sides\":[{\"content\":{\"connectorIds\":[\"In1\"]},\"type\":\"ConnectorPlacement.EquallySpacedRectSide\",\"uuid\":\"27fa7930-342b-464c-b74e-3dc50cf3e81b\"},{\"content\":{\"connectorIds\":[\"Out1\"],\"side\":\"RIGHT\"},\"type\":\"ConnectorPlacement.EquallySpacedRectSide\",\"uuid\":\"52054d8e-df5f-449a-98bd-11d1376604f8\"},{\"content\":{\"side\":\"TOP\"},\"type\":\"ConnectorPlacement.EquallySpacedRectSide\",\"uuid\":\"b1419e4b-fc7c-4452-8b54-b25730e7b81d\"},{\"content\":{\"connectorIds\":[\"In2\"],\"side\":\"BOTTOM\"},\"type\":\"ConnectorPlacement.EquallySpacedRectSide\",\"uuid\":\"7ca70ec0-7c1b-4387-990e-8fb77f2b010c\"}]},\"type\":\"ConnectorPlacement.EquallySpacedConnector\",\"uuid\":\"6a86a2d4-e98f-4743-adb4-c0b70975b9c2\"}],\"packageUris\":[\"http://schema.mathworks.com/mf0/Connector/R2020b\"],\"version\":\"1.0\"}"
  Constant : Constant  Value=Lambda_matrix
  Gain : Gain  Gain=F_matrix  Multiplication=Matrix(K*u)
  MatrixMultiply : Product  Multiplication=Matrix(*)
  Product : Product  Multiplication=Matrix(*)
  Step : Step  Time=0  Before=diag([0, 0, 0, 0, 0, 0])  After=0*eye(6)  SampleTime=0
  Sum : Sum  Inputs=|+-
  Transpose : Math  Operator=transpose
  Thrust_forces : Outport
  wires:
  tau_c/1 -> Allocation/2(tau_c)
  Allocation/1(Omega_cmd) -> Actuator Dynamics/1(Omega_cmd)  "Omega_cmd"
  Product/1 -> Allocation/1(T_c)
  Transpose/1 -> Product/1
  R/1 -> Transpose/1
  T_c/1 -> Product/2
  Sum/1 -> MatrixMultiply/1
  Constant/1 -> Sum/1
  Step/1 -> Sum/2
  Gain/1 -> Thrust_forces/1
  Actuator Dynamics/1(Thrust_forces) -> MatrixMultiply/2
  MatrixMultiply/1 -> Gain/1

== system RB_dyn/Atittude Planner & Controller ==
  fc_i : Inport
  R : Inport  Port=2
  psi_d : Inport  Port=3
  omega : Inport  Port=4
  Atittude Controller : Subsystem
      settings: PortSchema="{\"entries\":[{\"content\":{\"sides\":[{\"content\":{\"connectorIds\":[\"In1\",\"In2\",\"In3\"]},\"type\":\"ConnectorPlacement.EquallySpacedRectSide\",\"uuid\":\"45854091-1ad4-48de-a2c2-5228965603de\"},{\"content\":{\"side\":\"RIGHT\"},\"type\":\"ConnectorPlacement.EquallySpacedRectSide\",\"uuid\":\"a293c214-bcaa-4f60-a42a-539eda776e35\"},{\"content\":{\"connectorIds\":[\"Out1\"],\"side\":\"TOP\"},\"type\":\"ConnectorPlacement.EquallySpacedRectSide\",\"uuid\":\"6a2ea071-b3c4-435f-ab31-1c30f1e1fcfe\"}]},\"type\":\"ConnectorPlacement.EquallySpacedConnector\",\"uuid\":\"defa2961-a4c8-4cfa-8923-ba6f5f73b83c\"}],\"packageUris\":[\"http://schema.mathworks.com/mf0/Connector/R2020b\"],\"version\":\"1.0\"}"
  Atittude Planner : Subsystem
      settings: PortSchema="{\"entries\":[{\"content\":{\"sides\":[{\"content\":{\"connectorIds\":[\"In1\"]},\"type\":\"ConnectorPlacement.EquallySpacedRectSide\",\"uuid\":\"45854091-1ad4-48de-a2c2-5228965603de\"},{\"content\":{\"connectorIds\":[\"Out1\"],\"side\":\"RIGHT\"},\"type\":\"ConnectorPlacement.EquallySpacedRectSide\",\"uuid\":\"a293c214-bcaa-4f60-a42a-539eda776e35\"},{\"content\":{\"connectorIds\":[\"In2\"],\"side\":\"TOP\"},\"type\":\"ConnectorPlacement.EquallySpacedRectSide\",\"uuid\":\"6a2ea071-b3c4-435f-ab31-1c30f1e1fcfe\"}]},\"type\":\"ConnectorPlacement.EquallySpacedConnector\",\"uuid\":\"defa2961-a4c8-4cfa-8923-ba6f5f73b83c\"}],\"packageUris\":[\"http://schema.mathworks.com/mf0/Connector/R2020b\"],\"version\":\"1.0\"}"
  tau_c : Outport
  wires:
  Atittude Planner/1(R_d) -> Atittude Controller/1(R_d)
  fc_i/1 -> Atittude Planner/2(fc_i)
  R/1 -> Atittude Controller/2(R)
  psi_d/1 -> Atittude Planner/1(psi_d)
  Atittude Controller/1(tau_c) -> tau_c/1
  omega/1 -> Atittude Controller/3(omega)

== system RB_dyn/Dinámica UAV ==
  Thrust : Inport
  Aerodynamic Damping : MATLAB Function  TreatAsAtomicUnit=on
  Gravity wrench : MATLAB Function  TreatAsAtomicUnit=on
  MATLAB Function : MATLAB Function  TreatAsAtomicUnit=on
  Matrix Divide : Product  Inputs=/*  Multiplication=Matrix(*)
  "Rigid Body dynamics&kinematics " : Subsystem
  Sum : Sum  Inputs=|+--
  p : Outport
  omegab : Outport  Port=2
  wires:
  Gravity wrench/1(w_g) -> Sum/3
  Sum/1 -> "Rigid Body dynamics&kinematics "/1(w_b)
  Aerodynamic Damping/1(D) -> Sum/2
  "Rigid Body dynamics&kinematics "/1(p) -> p/1
  "Rigid Body dynamics&kinematics "/3(vb) -> Aerodynamic Damping/1(v_b)
  "Rigid Body dynamics&kinematics "/4(omegab) -> Aerodynamic Damping/2(omega_b), omegab/1
  Thrust/1 -> Sum/1
  "Rigid Body dynamics&kinematics "/2(R) -> Matrix Divide/1, Gravity wrench/1(R)
  [p_i] -> MATLAB Function/1(p_i)
  MATLAB Function/1(vw) -> Matrix Divide/2
  Matrix Divide/1 -> Aerodynamic Damping/3(vw)

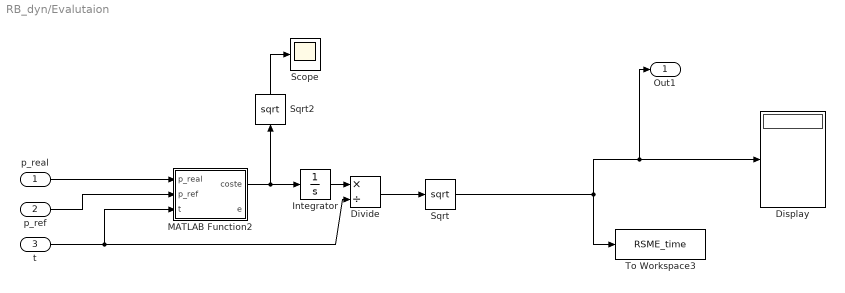
== system RB_dyn/Evalutaion ==
  p_real : Inport
  p_ref : Inport  Port=2
  t : Inport  Port=3
  Display : Display
  Divide : Product  Inputs=*/
  Integrator : Integrator
  MATLAB Function2 : MATLAB Function  TreatAsAtomicUnit=on
  Scope : Scope
  Sqrt : Sqrt  OutputSignalType=complex
  Sqrt2 : Sqrt
  To Workspace3 : ToWorkspace  VariableName=RSME_time  SaveFormat=Timeseries  SampleTime=-1
  Out1 : Outport
  wires:
  Divide/1 -> Sqrt/1
  MATLAB Function2/1(coste) -> Sqrt2/1, Integrator/1
  Sqrt/1 -> To Workspace3/1, Out1/1, Display/1
  p_ref/1 -> MATLAB Function2/2(p_ref)
  t/1 -> MATLAB Function2/3(t), Divide/2
  p_real/1 -> MATLAB Function2/1(p_real)
  Integrator/1 -> Divide/1
  Sqrt2/1 -> Scope/1

== system RB_dyn/Position Controller ==
  p : Inport
  p_d : Inport  Port=2
  v : Inport  Port=3
  " V Controller" : Subsystem
  Constant : Constant  Commented=on  Value=par.g*par.e_3
  Gain : Gain  Commented=on  Gain=m_t_est
  Pos Controller : Subsystem
      settings: PortSchema="{\"entries\":[{\"content\":{\"sides\":[{\"content\":{},\"type\":\"ConnectorPlacement.EquallySpacedRectSide\",\"uuid\":\"2fb879fa-9caa-4b67-ad1c-6d77d0280c38\"},{\"content\":{\"connectorIds\":[\"Out1\"],\"side\":\"RIGHT\"},\"type\":\"ConnectorPlacement.EquallySpacedRectSide\",\"uuid\":\"82fa2ff9-e48a-4751-98bb-12047787667e\"},{\"content\":{\"side\":\"TOP\"},\"type\":\"ConnectorPlacement.EquallySpacedRectSide\",\"uuid\":\"70e781bb-fb0f-473c-82a2-e9ed483c0d65\"},{\"content\":{\"connectorIds\":[\"In1\",\"In2\"],\"side\":\"BOTTOM\"},\"type\":\"ConnectorPlacement.EquallySpacedRectSide\",\"uuid\":\"1bc1f217-6b4c-4a6c-b3cf-0622d8ade2ed\"}]},\"type\":\"ConnectorPlacement.EquallySpacedConnector\",\"uuid\":\"d006ffe8-6230-4662-ba3a-e7870a3b1b43\"}],\"packageUris\":[\"http://schema.mathworks.com/mf0/Connector/R2020b\"],\"version\":\"1.0\"}"
  Sum : Sum  Inputs=|++
  fc_i : Outport
  wires:
  p_d/1 -> Pos Controller/1(p_cmd)
  Pos Controller/1(v_cmd) -> " V Controller"/1(v_cmd)
  v/1 -> " V Controller"/2(v)
  p/1 -> Pos Controller/2(p)
  " V Controller"/1(u_bl) -> Sum/1
  Constant/1 -> Gain/1
  Gain/1 -> Sum/2
  Sum/1 -> fc_i/1

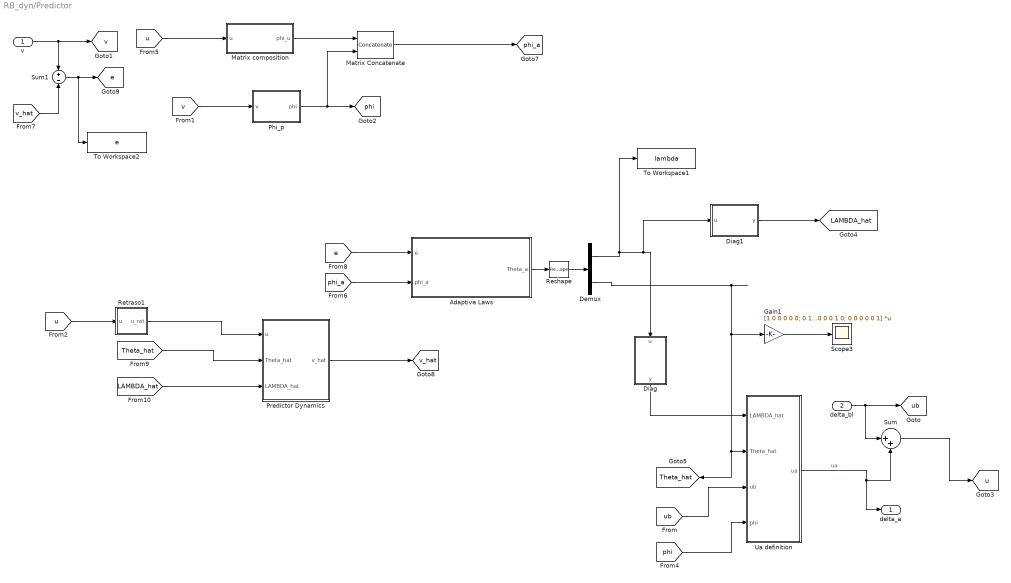
== system RB_dyn/Predictor ==
  v : Inport
  delta_bl : Inport  Port=2
  Adaptive Laws : Subsystem
  Demux : Demux  Outputs=[3,6]
  Diag : MATLAB Function  TreatAsAtomicUnit=on
  Diag1 : MATLAB Function  TreatAsAtomicUnit=on
  Gain1 : Gain  Gain=[1 0 0 0 0 0; 0 1 0 0 0 0;0 0 0 1 0 0; 0 0 0 0 1 0; 0 0 0 0 0 1]  Multiplication=Matrix(K*u)
  Matrix Concatenate : Concatenate  Mode=Multidimensional array
  Matrix composition : Subsystem
  Phi_p : MATLAB Function  TreatAsAtomicUnit=on
  Predictor Dynamics : Subsystem
  Reshape : Reshape  OutputDimensionality=Column vector (2-D)
  Retraso1 : Subsystem
  Scope3 : Scope
  Sum : Sum  Inputs=|++
  Sum1 : Sum  Inputs=+-
  To Workspace1 : ToWorkspace  VariableName=lambda  SaveFormat=Timeseries  SampleTime=-1
  To Workspace2 : ToWorkspace  VariableName=e  SaveFormat=Timeseries  SampleTime=-1
  Ua definition : Subsystem
  delta_a : Outport  PortDimensions=[3,1]
  tag scope: LAMBDA_hat=global, Theta_hat=global, e=global, phi=global, phi_a=global, u=global, ub=global, v=global, v_hat=global
  wires:
  Ua definition/1(ua) -> delta_a/1, Sum/2  "ua"
  Sum/1 -> [u]
  delta_bl/1 -> [ub], Sum/1
  v/1 -> Sum1/1, [v]
  [ub] -> Ua definition/3(ub)
  [v] -> Phi_p/1(v)
  Phi_p/1(phi) -> Matrix Concatenate/2, [phi]
  [u] -> Retraso1/1(u)
  [phi] -> Ua definition/4(phi)
  Adaptive Laws/1(Theta_a) -> Reshape/1
  Demux/1 -> Diag/1(u), Diag1/1(u), To Workspace1/1
  Matrix Concatenate/1 -> [phi_a]
  [phi_a] -> Adaptive Laws/2(phi_a)
  Predictor Dynamics/1(v_hat) -> [v_hat]
  [v_hat] -> Sum1/2
  Sum1/1 -> To Workspace2/1, [e]
  [e] -> Adaptive Laws/1(e)
  [Theta_hat] -> Predictor Dynamics/2(Theta_hat)
  [LAMBDA_hat] -> Predictor Dynamics/3(LAMBDA_hat)
  Demux/2 -> Gain1/1, [Theta_hat], Ua definition/2(Theta_hat)
  Matrix composition/1(phi_u) -> Matrix Concatenate/1
  Diag/1(y) -> Ua definition/1(LAMBDA_hat)
  Reshape/1 -> Demux/1
  Diag1/1(y) -> [LAMBDA_hat]
  Retraso1/1(u_ret) -> Predictor Dynamics/1(u)
  [u] -> Matrix composition/1(u)
  Gain1/1 -> Scope3/1

== system RB_dyn/Ts_pos_adapt1 ==
  tau : Inport
  1-D Lookup Table : Lookup_n-D  NumberOfTableDimensions=1  BreakpointsForDimension1=t_lookup  Table=p_x_data  ExtrapMethod=Clip  InternalRulePriority=Speed  RndMeth=Simplest
  1-D Lookup Table1 : Lookup_n-D  NumberOfTableDimensions=1  BreakpointsForDimension1=t_lookup  Table=p_y_data  ExtrapMethod=Clip  InternalRulePriority=Speed  RndMeth=Simplest
  1-D Lookup Table2 : Lookup_n-D  NumberOfTableDimensions=1  BreakpointsForDimension1=t_lookup  Table=p_z_data  ExtrapMethod=Clip  InternalRulePriority=Speed  RndMeth=Simplest
  Mux : Mux  Inputs=3
  p_d : Outport
  wires:
  tau/1 -> 1-D Lookup Table1/1, 1-D Lookup Table/1, 1-D Lookup Table2/1
  1-D Lookup Table/1 -> Mux/1
  1-D Lookup Table1/1 -> Mux/2
  1-D Lookup Table2/1 -> Mux/3
  Mux/1 -> p_d/1

== system RB_dyn/V limitation ==
  p_d : Inport
  Gain : Gain  Gain=K_position  Multiplication=Matrix(K*u)
  Scope : Scope
  Scope1 : Scope
  Sum : Sum  Inputs=+-
  V_limitation : MATLAB Function  TreatAsAtomicUnit=on
  v_cmd integrator : Integrator  InitialCondition=p_0
  p_cmd : Outport
  wires:
  p_d/1 -> Sum/1
  v_cmd integrator/1 -> Sum/2, p_cmd/1
  Sum/1 -> Scope1/1, Gain/1
  Gain/1 -> Scope/1, V_limitation/1(v_cmd0)
  V_limitation/1(v_cmd) -> v_cmd integrator/1

== system RB_dyn/Allocation + Actuator Dynamics/Actuator Dynamics ==
  Omega_cmd : Inport
  Dinámica Propeller : Subsystem
  Scope : Scope
  "Thrust Model " : Subsystem
  Thrust_forces : Outport
  wires:
  Omega_cmd/1 -> Dinámica Propeller/1(Omegas_cmd)
  Dinámica Propeller/1(Omegas) -> "Thrust Model "/1(Omegas)
  "Thrust Model "/1(Thrust) -> Scope/1, Thrust_forces/1

== system RB_dyn/Allocation + Actuator Dynamics/Allocation ==
  T_c : Inport
  tau_c : Inport  Port=2
  Display : Display
  Display1 : Display
  Gain : Gain  Gain=Finv  Multiplication=Matrix(K*u)
  MATLAB Function : MATLAB Function  TreatAsAtomicUnit=on
  Mux : Mux  Inputs=2
  Saturacion : Saturate  UpperLimit=(k_f*UAV.Omega_max^2)*ones(6,1)  LowerLimit=(k_f*UAV.Omega_min^2)*ones(6,1)
  Scope : Scope
  Omega_cmd : Outport
  wires:
  T_c/1 -> Mux/1
  tau_c/1 -> Mux/2
  Mux/1 -> Gain/1
  Gain/1 -> Saturacion/1
  MATLAB Function/1(Omega) -> Display1/1, Scope/1, Omega_cmd/1
  Saturacion/1 -> Display/1, MATLAB Function/1(T)

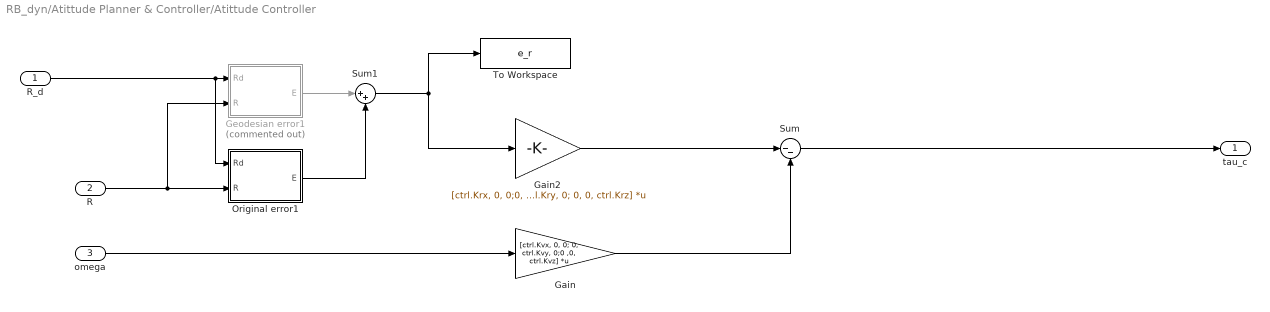
== system RB_dyn/Atittude Planner & Controller/Atittude Controller ==
  R_d : Inport
  R : Inport  Port=2
  omega : Inport  Port=3
  Gain : Gain  Gain=[ctrl.Kvx, 0, 0; 0, ctrl.Kvy, 0;0 ,0, ctrl.Kvz]  Multiplication=Matrix(K*u)
  Gain2 : Gain  Gain=[ctrl.Krx, 0, 0;0, ctrl.Kry, 0; 0, 0, ctrl.Krz]  Multiplication=Matrix(K*u)
  Geodesian error1 : MATLAB Function  Commented=on  TreatAsAtomicUnit=on
  Original error1 : MATLAB Function  TreatAsAtomicUnit=on
  Sum : Sum  Inputs=|--
  Sum1 : Sum  Inputs=|++
  To Workspace : ToWorkspace  VariableName=e_r  SaveFormat=Timeseries  SampleTime=-1
  tau_c : Outport
  wires:
  omega/1 -> Gain/1
  Gain2/1 -> Sum/1
  R_d/1 -> Original error1/1(Rd), Geodesian error1/1(Rd)
  Sum/1 -> tau_c/1
  Gain/1 -> Sum/2
  R/1 -> Original error1/2(R), Geodesian error1/2(R)
  Geodesian error1/1(E) -> Sum1/1
  Original error1/1(E) -> Sum1/2
  Sum1/1 -> Gain2/1, To Workspace/1

== system RB_dyn/Atittude Planner & Controller/Atittude Planner ==
  psi_d : Inport
  fc_i : Inport  Port=2
  Display : Display
  Display1 : Display
  Display2 : Display
  MATLAB Function : MATLAB Function  TreatAsAtomicUnit=on
  MATLAB Function1 : MATLAB Function  TreatAsAtomicUnit=on
  MATLAB Function2 : MATLAB Function  TreatAsAtomicUnit=on
  Matrix Concatenate : Concatenate  NumInputs=3  Mode=Multidimensional array  ConcatenateDimension=2
  R_d : Outport
  wires:
  fc_i/1 -> MATLAB Function/1(fc)
  MATLAB Function/1(kp) -> Display1/1, Matrix Concatenate/3, MATLAB Function2/1(kp)
  MATLAB Function1/1(hd) -> MATLAB Function2/2(hd), Display2/1
  Matrix Concatenate/1 -> Display/1, R_d/1
  MATLAB Function2/2(jp) -> Matrix Concatenate/2
  MATLAB Function2/1(ip) -> Matrix Concatenate/1
  psi_d/1 -> MATLAB Function1/1(psi_d)

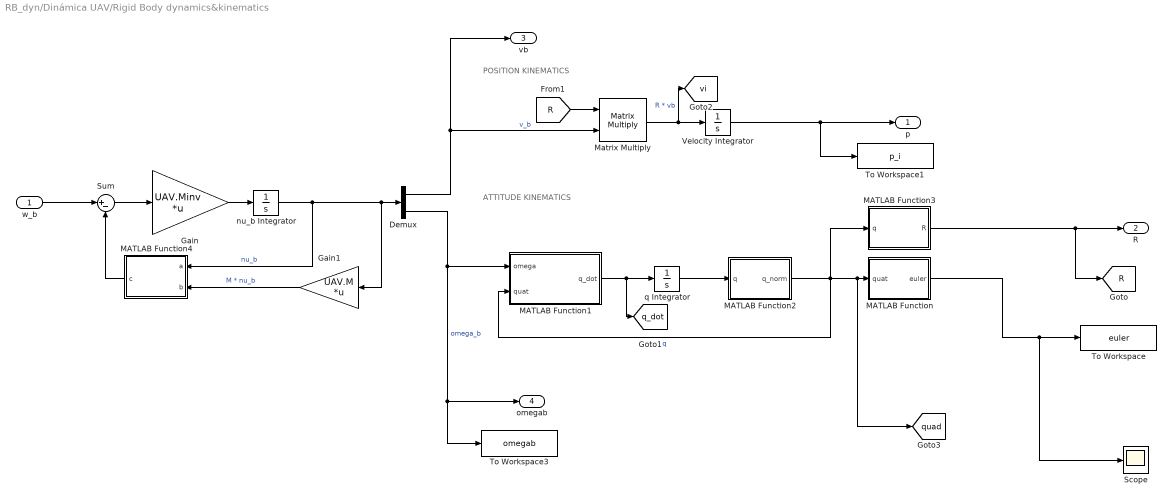
== system RB_dyn/Dinámica UAV/Rigid Body dynamics&kinematics  ==
  note: ATTITUDE KINEMATICS
  note: POSITION KINEMATICS
  w_b : Inport
  Demux : Demux  Outputs=2
  Gain : Gain  Gain=UAV.Minv  Multiplication=Matrix(K*u)
  Gain1 : Gain  Gain=UAV.M  Multiplication=Matrix(K*u)
  MATLAB Function : MATLAB Function  TreatAsAtomicUnit=on
  MATLAB Function1 : MATLAB Function  TreatAsAtomicUnit=on
  MATLAB Function2 : MATLAB Function  TreatAsAtomicUnit=on
  MATLAB Function3 : MATLAB Function  TreatAsAtomicUnit=on
  MATLAB Function4 : MATLAB Function  TreatAsAtomicUnit=on
  Matrix Multiply : Product  Multiplication=Matrix(*)
  Scope : Scope
  Sum : Sum  Inputs=|+-
  To Workspace : ToWorkspace  VariableName=euler  SaveFormat=Timeseries  SampleTime=-1
  To Workspace1 : ToWorkspace  VariableName=p_i  SaveFormat=Timeseries  SampleTime=-1
  To Workspace3 : ToWorkspace  VariableName=omegab  SaveFormat=Timeseries  SampleTime=-1
  Velocity Integrator : Integrator  InitialCondition=p_0
  nu_b Integrator : Integrator  InitialCondition=[vb_0;omegab_0]
  q Integrator : Integrator  InitialCondition=q_0
  p : Outport
  R : Outport  Port=2
  vb : Outport  Port=3
  omegab : Outport  Port=4
  tag scope: R=global, q_dot=global, quad=global, vi=global
  wires:
  Velocity Integrator/1 -> p/1, To Workspace1/1
  MATLAB Function1/1(q_dot) -> [q_dot], q Integrator/1
  MATLAB Function2/1(q_norm) -> MATLAB Function3/1(q), MATLAB Function1/2(quat), [quad], MATLAB Function/1(quat)  "q"
  MATLAB Function3/1(R) -> R/1, [R]
  Demux/1 -> vb/1, Matrix Multiply/2  "v_b"
  nu_b Integrator/1 -> Demux/1, Gain1/1, MATLAB Function4/1(a)  "nu_b"
  q Integrator/1 -> MATLAB Function2/1(q)
  Matrix Multiply/1 -> [vi], Velocity Integrator/1  "R * vb"
  MATLAB Function/1(euler) -> Scope/1, To Workspace/1
  [R] -> Matrix Multiply/1
  Gain/1 -> nu_b Integrator/1
  Demux/2 -> omegab/1, To Workspace3/1, MATLAB Function1/1(omega)  "omega_b"
  Gain1/1 -> MATLAB Function4/2(b)  "M * nu_b"
  Sum/1 -> Gain/1
  MATLAB Function4/1(c) -> Sum/2
  w_b/1 -> Sum/1

== system RB_dyn/Position Controller/ V Controller ==
  v_cmd : Inport
  v : Inport  Port=2
  Gain : Gain  Gain=Ki  Multiplication=Matrix(K*u)
  Gain1 : Gain  Gain=Kp  Multiplication=Matrix(K*u)
  Sum : Sum  Inputs=+-
  Sum1 : Sum
  ev integrator : Integrator  InitialCondition=zeros(3,1)
  u_bl : Outport
  wires:
  v/1 -> Sum/2
  v_cmd/1 -> Sum/1
  Sum/1 -> Gain1/1, ev integrator/1
  ev integrator/1 -> Gain/1
  Gain1/1 -> Sum1/2
  Gain/1 -> Sum1/1
  Sum1/1 -> u_bl/1

== system RB_dyn/Position Controller/Pos Controller ==
  p_cmd : Inport
  p : Inport  Port=2
  Clock : Clock
  Divide : Product  Inputs=*/
  Gain : Gain  Gain=K_position  Multiplication=Matrix(K*u)
  Integrator : Integrator
  MATLAB Function2 : MATLAB Function  TreatAsAtomicUnit=on
  Scope : Scope
  Sum : Sum  Inputs=+-
  mean d : Display
  v_cmd : Outport
  wires:
  Sum/1 -> MATLAB Function2/1(u), Gain/1
  Gain/1 -> v_cmd/1
  p/1 -> Sum/2
  p_cmd/1 -> Sum/1
  MATLAB Function2/1(y) -> Integrator/1, Scope/1
  Integrator/1 -> Divide/1
  Clock/1 -> Divide/2
  Divide/1 -> mean d/1

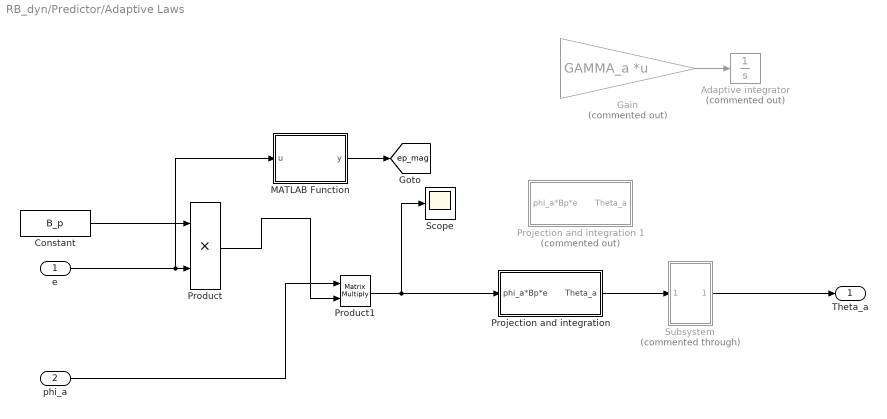
== system RB_dyn/Predictor/Adaptive Laws ==
  e : Inport
  phi_a : Inport  Port=2
  Adaptive integrator : Integrator  Commented=on  InitialCondition=[LAMBDA_hat_0;Theta_0]
  Constant : Constant  Value=B_p
  Gain : Gain  Commented=on  Gain=GAMMA_a  Multiplication=Matrix(K*u)
  MATLAB Function : MATLAB Function  TreatAsAtomicUnit=on
  Product : Product
  Product1 : Product  Multiplication=Matrix(*)
  "Projection and integration " : Subsystem
  Projection and integration 1 : Subsystem  Commented=on
  Scope : Scope
  Subsystem : Subsystem  Commented=through
  Theta_a : Outport  PortDimensions=[9,1]
  tag scope: ep_mag=global
  wires:
  e/1 -> MATLAB Function/1(u), Product/2
  Constant/1 -> Product/1
  Product/1 -> Product1/2
  Gain/1 -> Adaptive integrator/1
  phi_a/1 -> Product1/1
  Product1/1 -> "Projection and integration "/1(phi_a*Bp*e), Scope/1
  "Projection and integration "/1(Theta_a) -> Subsystem/1(In1)
  Subsystem/1(Out1) -> Theta_a/1
  MATLAB Function/1(y) -> [ep_mag]

== system RB_dyn/Predictor/Matrix composition ==
  u : Inport
  Demux : Demux  Outputs=3
  Gain : Gain  Gain=[1 ,0, 0]  Multiplication=Matrix(u*K)
  Gain1 : Gain  Gain=[0, 1, 0]  Multiplication=Matrix(u*K)
  Gain2 : Gain  Gain=[0, 0, 1]  Multiplication=Matrix(u*K)
  Matrix Concatenate : Concatenate  NumInputs=3  Mode=Multidimensional array
  phi_u : Outport  PortDimensions=[3,3]
  wires:
  u/1 -> Demux/1
  Demux/1 -> Gain/1
  Demux/3 -> Gain2/1
  Demux/2 -> Gain1/1
  Gain/1 -> Matrix Concatenate/1
  Gain1/1 -> Matrix Concatenate/2
  Gain2/1 -> Matrix Concatenate/3
  Matrix Concatenate/1 -> phi_u/1

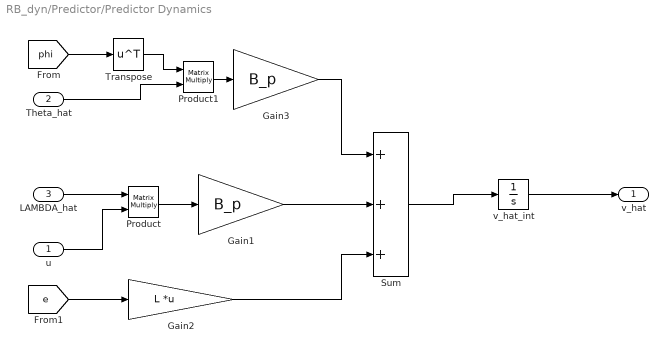
== system RB_dyn/Predictor/Predictor Dynamics ==
  u : Inport
  Theta_hat : Inport  Port=2  PortDimensions=[6,1]
  LAMBDA_hat : Inport  Port=3  PortDimensions=[3,3]
  Gain1 : Gain  Gain=B_p
  Gain2 : Gain  Gain=L  Multiplication=Matrix(K*u)
  Gain3 : Gain  Gain=B_p
  Product : Product  Multiplication=Matrix(*)
  Product1 : Product  Multiplication=Matrix(*)
  Sum : Sum  Inputs=+++
  Transpose : Math  Operator=transpose
  v_hat_int : Integrator  InitialCondition=v_0
  v_hat : Outport  PortDimensions=[3,1]
  wires:
  v_hat_int/1 -> v_hat/1
  Sum/1 -> v_hat_int/1
  Product/1 -> Gain1/1
  Gain1/1 -> Sum/2
  [phi] -> Transpose/1
  Theta_hat/1 -> Product1/2
  Transpose/1 -> Product1/1
  Product1/1 -> Gain3/1
  [e] -> Gain2/1
  Gain2/1 -> Sum/3
  Gain3/1 -> Sum/1
  LAMBDA_hat/1 -> Product/1
  u/1 -> Product/2

== system RB_dyn/Predictor/Retraso1 ==
  u : Inport
  Demux : Demux  Outputs=3
  Mux : Mux  Inputs=3
  Transfer Fcn : TransferFcn  Denominator=[0.15 1]
  Transfer Fcn1 : TransferFcn  Denominator=[0.15 1]
  Transfer Fcn2 : TransferFcn  Denominator=[0.15 1]
  u_ret : Outport
  wires:
  u/1 -> Demux/1
  Mux/1 -> u_ret/1
  Demux/1 -> Transfer Fcn/1
  Transfer Fcn/1 -> Mux/1
  Demux/2 -> Transfer Fcn1/1
  Transfer Fcn1/1 -> Mux/2
  Demux/3 -> Transfer Fcn2/1
  Transfer Fcn2/1 -> Mux/3

== system RB_dyn/Predictor/Ua definition ==
  LAMBDA_hat : Inport
  Theta_hat : Inport  Port=2  PortDimensions=[6,1]
  ub : Inport  Port=3
  phi : Inport  Port=4
  Matrix Divide : Product  Inputs=/*  Multiplication=Matrix(*)
  Matrix Divide1 : Product  Inputs=/*  Multiplication=Matrix(*)
  Product : Product  Multiplication=Matrix(*)
  Sum : Sum  Inputs=-+-
  Transpose : Math  Operator=transpose
  ua : Outport  PortDimensions=[3,1]
  wires:
  Sum/1 -> ua/1
  ub/1 -> Matrix Divide/2, Sum/1
  Matrix Divide/1 -> Sum/2
  LAMBDA_hat/1 -> Matrix Divide1/1, Matrix Divide/1
  phi/1 -> Transpose/1
  Matrix Divide1/1 -> Sum/3
  Transpose/1 -> Product/1
  Theta_hat/1 -> Product/2
  Product/1 -> Matrix Divide1/2

== system RB_dyn/Allocation + Actuator Dynamics/Actuator Dynamics/Dinámica Propeller ==
  Omegas_cmd : Inport
  Gain : Gain  Gain=-UAV.k_m
  Integrator : Integrator  InitialCondition=UAV.Omega_0*ones(6,1)
  Sum : Sum  Inputs=|+-
  Omegas : Outport
  wires:
  Omegas_cmd/1 -> Sum/2
  Sum/1 -> Gain/1
  Integrator/1 -> Omegas/1, Sum/1
  Gain/1 -> Integrator/1

== system RB_dyn/Allocation + Actuator Dynamics/Actuator Dynamics/Thrust Model  ==
  Omegas : Inport
  Dinamica : MATLAB Function  TreatAsAtomicUnit=on
  Saturacion : Saturate  UpperLimit=UAV.Omega_max*ones(6,1)  LowerLimit=UAV.Omega_min*ones(6,1)
  Scope : Scope
  Thrust : Outport
  wires:
  Dinamica/1(T_arg) -> Thrust/1
  Omegas/1 -> Saturacion/1
  Saturacion/1 -> Scope/1, Dinamica/1(Omegas)

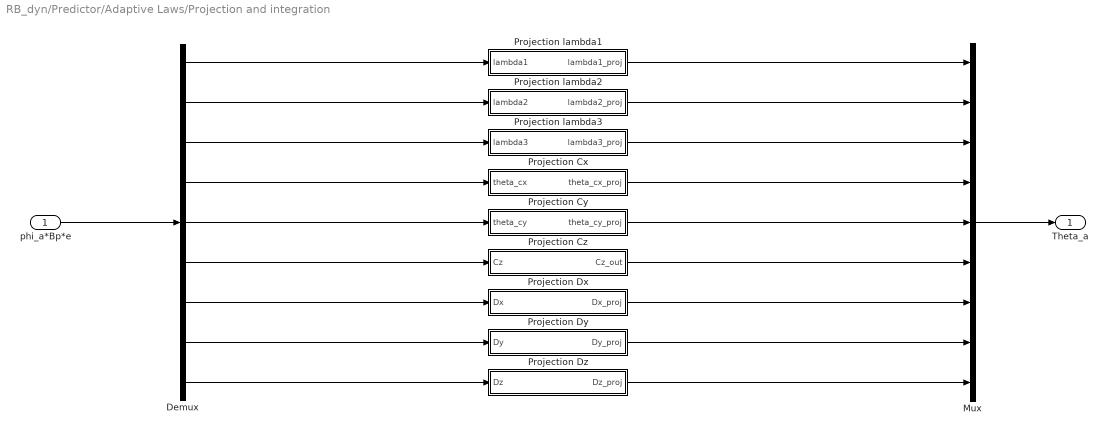
== system RB_dyn/Predictor/Adaptive Laws/Projection and integration  ==
  phi_a*Bp*e : Inport
  Demux : Demux  Outputs=9
  Mux : Mux  Inputs=9
  Projection Cx : Subsystem
  Projection Cy : Subsystem
  Projection Cz : Subsystem
  Projection Dx : Subsystem
  Projection Dy : Subsystem
  Projection Dz : Subsystem
  Projection lambda1 : Subsystem
  Projection lambda2 : Subsystem
  Projection lambda3 : Subsystem
  Theta_a : Outport
  wires:
  phi_a*Bp*e/1 -> Demux/1
  Demux/1 -> Projection lambda1/1(lambda1)
  Projection lambda1/1(lambda1_proj) -> Mux/1
  Demux/2 -> Projection lambda2/1(lambda2)
  Projection lambda2/1(lambda2_proj) -> Mux/2
  Demux/3 -> Projection lambda3/1(lambda3)
  Projection lambda3/1(lambda3_proj) -> Mux/3
  Demux/4 -> Projection Cx/1(theta_cx)
  Projection Cx/1(theta_cx_proj) -> Mux/4
  Demux/5 -> Projection Cy/1(theta_cy)
  Projection Cy/1(theta_cy_proj) -> Mux/5
  Demux/6 -> Projection Cz/1(Cz)
  Projection Cz/1(Cz_out) -> Mux/6
  Demux/7 -> Projection Dx/1(Dx)
  Projection Dx/1(Dx_proj) -> Mux/7
  Demux/8 -> Projection Dy/1(Dy)
  Projection Dy/1(Dy_proj) -> Mux/8
  Demux/9 -> Projection Dz/1(Dz)
  Projection Dz/1(Dz_proj) -> Mux/9
  Mux/1 -> Theta_a/1

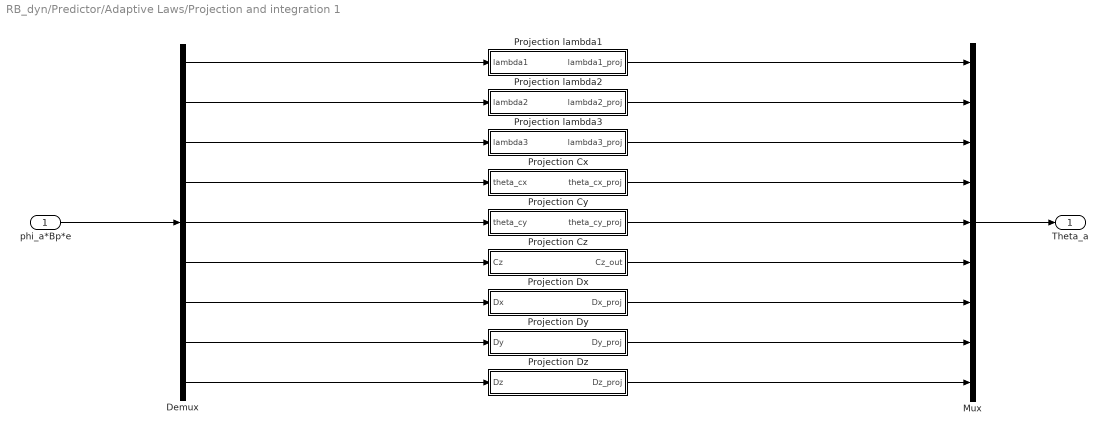
== system RB_dyn/Predictor/Adaptive Laws/Projection and integration 1 ==
  phi_a*Bp*e : Inport
  Demux : Demux  Outputs=9
  Mux : Mux  Inputs=9
  Projection Cx : Subsystem
  Projection Cy : Subsystem
  Projection Cz : Subsystem
  Projection Dx : Subsystem
  Projection Dy : Subsystem
  Projection Dz : Subsystem
  Projection lambda1 : Subsystem
  Projection lambda2 : Subsystem
  Projection lambda3 : Subsystem
  Theta_a : Outport
  wires:
  phi_a*Bp*e/1 -> Demux/1
  Demux/1 -> Projection lambda1/1(lambda1)
  Projection lambda1/1(lambda1_proj) -> Mux/1
  Demux/2 -> Projection lambda2/1(lambda2)
  Projection lambda2/1(lambda2_proj) -> Mux/2
  Demux/3 -> Projection lambda3/1(lambda3)
  Projection lambda3/1(lambda3_proj) -> Mux/3
  Demux/4 -> Projection Cx/1(theta_cx)
  Projection Cx/1(theta_cx_proj) -> Mux/4
  Demux/5 -> Projection Cy/1(theta_cy)
  Projection Cy/1(theta_cy_proj) -> Mux/5
  Demux/6 -> Projection Cz/1(Cz)
  Projection Cz/1(Cz_out) -> Mux/6
  Demux/7 -> Projection Dx/1(Dx)
  Projection Dx/1(Dx_proj) -> Mux/7
  Demux/8 -> Projection Dy/1(Dy)
  Projection Dy/1(Dy_proj) -> Mux/8
  Demux/9 -> Projection Dz/1(Dz)
  Projection Dz/1(Dz_proj) -> Mux/9
  Mux/1 -> Theta_a/1

== system RB_dyn/Predictor/Adaptive Laws/Subsystem ==
  In1 : Inport
  Gain1 : Gain  Gain=GAMMA_a  Multiplication=Matrix(K*u)
  Integrator : Integrator  InitialCondition=[LAMBDA_hat_0;Theta_0]
  Out1 : Outport
  wires:
  Gain1/1 -> Integrator/1
  In1/1 -> Gain1/1
  Integrator/1 -> Out1/1

== system RB_dyn/Predictor/Adaptive Laws/Projection and integration /Projection Cx ==
  theta_cx : Inport
  Constant : Constant  Value=proj.CenterCxy
  Gain : Gain  Gain=proj.sigma
  Integrator : Integrator  InitialCondition=Theta_0(1) - proj.CenterCxy
  Product : Product
  Projection : MATLAB Function  TreatAsAtomicUnit=on
  Sum : Sum
  Sum1 : Sum  Inputs=|+-
  Sum2 : Sum  Inputs=|+-
  theta_cx_proj : Outport
  wires:
  Integrator/1 -> Sum2/1, Sum/2
  Constant/1 -> Sum2/2, Sum/1
  Sum/1 -> theta_cx_proj/1, Projection/1(theta)
  theta_cx/1 -> Sum1/1
  Sum1/1 -> Projection/2(y)
  [ep_mag] -> Product/2
  Sum2/1 -> Product/1
  Product/1 -> Gain/1
  Gain/1 -> Sum1/2
  Projection/1(y_proj) -> Integrator/1

== system RB_dyn/Predictor/Adaptive Laws/Projection and integration /Projection Cy ==
  theta_cy : Inport
  Constant : Constant  Value=proj.CenterCxy
  Gain : Gain  Gain=proj.sigma
  Integrator : Integrator  InitialCondition=Theta_0(2) - proj.CenterCxy
  Product : Product
  Projection : MATLAB Function  TreatAsAtomicUnit=on
  Sum : Sum
  Sum1 : Sum  Inputs=|+-
  Sum2 : Sum  Inputs=|+-
  theta_cy_proj : Outport
  wires:
  Sum/1 -> theta_cy_proj/1, Projection/1(theta)
  Gain/1 -> Sum1/2
  Constant/1 -> Sum2/2, Sum/1
  Sum2/1 -> Product/1
  Integrator/1 -> Sum2/1, Sum/2
  [ep_mag] -> Product/2
  Product/1 -> Gain/1
  theta_cy/1 -> Sum1/1
  Sum1/1 -> Projection/2(y)
  Projection/1(y_proj) -> Integrator/1

== system RB_dyn/Predictor/Adaptive Laws/Projection and integration /Projection Cz ==
  Cz : Inport
  Gain : Gain  Gain=GAMMA_a(6,6)
  Integrator : Integrator  InitialCondition=Theta_0(3)
  Cz_out : Outport
  wires:
  Cz/1 -> Gain/1
  Integrator/1 -> Cz_out/1
  Gain/1 -> Integrator/1

== system RB_dyn/Predictor/Adaptive Laws/Projection and integration /Projection Dx ==
  Dx : Inport
  Constant : Constant  Value=proj.CenterDxy
  Gain : Gain  Gain=proj.sigma
  Integrator : Integrator  InitialCondition=Theta_0(4) - proj.CenterDxy
  Product : Product
  Projection : MATLAB Function  TreatAsAtomicUnit=on
  Sum : Sum
  Sum1 : Sum  Inputs=|+-
  Sum2 : Sum  Inputs=|+-
  Dx_proj : Outport
  wires:
  Sum/1 -> Dx_proj/1, Projection/1(theta)
  Gain/1 -> Sum1/2
  Constant/1 -> Sum2/2, Sum/1
  Sum2/1 -> Product/1
  Integrator/1 -> Sum2/1, Sum/2
  [ep_mag] -> Product/2
  Product/1 -> Gain/1
  Dx/1 -> Sum1/1
  Sum1/1 -> Projection/2(y)
  Projection/1(y_proj) -> Integrator/1

== system RB_dyn/Predictor/Adaptive Laws/Projection and integration /Projection Dy ==
  Dy : Inport
  Constant : Constant  Value=proj.CenterDxy
  Gain : Gain  Gain=proj.sigma
  Integrator : Integrator  InitialCondition=Theta_0(5) - proj.CenterDxy
  Product : Product
  Projection : MATLAB Function  TreatAsAtomicUnit=on
  Sum : Sum
  Sum1 : Sum  Inputs=|+-
  Sum2 : Sum  Inputs=|+-
  Dy_proj : Outport
  wires:
  Sum/1 -> Dy_proj/1, Projection/1(theta)
  Gain/1 -> Sum1/2
  Constant/1 -> Sum2/2, Sum/1
  Sum2/1 -> Product/1
  Integrator/1 -> Sum2/1, Sum/2
  [ep_mag] -> Product/2
  Product/1 -> Gain/1
  Dy/1 -> Sum1/1
  Sum1/1 -> Projection/2(y)
  Projection/1(y_proj) -> Integrator/1

== system RB_dyn/Predictor/Adaptive Laws/Projection and integration /Projection Dz ==
  Dz : Inport
  Constant : Constant  Value=proj.CenterDz
  Gain : Gain  Gain=proj.sigma
  Integrator : Integrator  InitialCondition=Theta_0(6) - proj.CenterDz
  Product : Product
  Projection : MATLAB Function  TreatAsAtomicUnit=on
  Sum : Sum
  Sum1 : Sum  Inputs=|+-
  Sum2 : Sum  Inputs=|+-
  Dz_proj : Outport
  wires:
  Sum/1 -> Dz_proj/1, Projection/1(theta)
  Gain/1 -> Sum1/2
  Constant/1 -> Sum2/2, Sum/1
  Sum2/1 -> Product/1
  Integrator/1 -> Sum2/1, Sum/2
  [ep_mag] -> Product/2
  Product/1 -> Gain/1
  Dz/1 -> Sum1/1
  Sum1/1 -> Projection/2(y)
  Projection/1(y_proj) -> Integrator/1

== system RB_dyn/Predictor/Adaptive Laws/Projection and integration /Projection lambda1 ==
  lambda1 : Inport
  Constant : Constant  Value=proj.CenterLambda
  Gain : Gain  Gain=proj.sigma
  Integrator : Integrator  InitialCondition=LAMBDA_hat_0(1) - proj.CenterLambda
  Product : Product
  Projection : MATLAB Function  TreatAsAtomicUnit=on
  Sum : Sum
  Sum1 : Sum  Inputs=+-
  Sum2 : Sum  Inputs=+-
  lambda1_proj : Outport
  wires:
  lambda1/1 -> Sum1/1
  Integrator/1 -> Sum2/1, Sum/2
  Constant/1 -> Sum2/2, Sum/1
  Gain/1 -> Sum1/2
  Sum1/1 -> Projection/2(y)
  Product/1 -> Gain/1
  [ep_mag] -> Product/2
  Sum2/1 -> Product/1
  Sum/1 -> lambda1_proj/1, Projection/1(theta)
  Projection/1(y_proj) -> Integrator/1

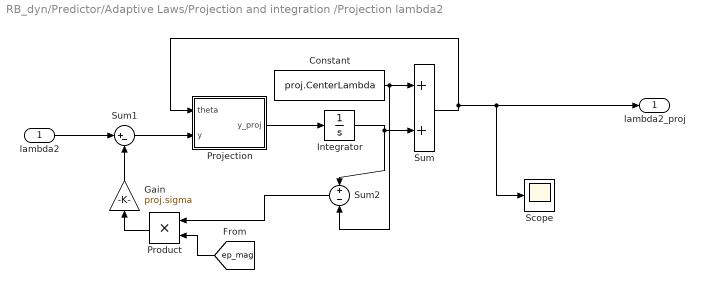
== system RB_dyn/Predictor/Adaptive Laws/Projection and integration /Projection lambda2 ==
  lambda2 : Inport
  Constant : Constant  Value=proj.CenterLambda
  Gain : Gain  Gain=proj.sigma
  Integrator : Integrator  InitialCondition=LAMBDA_hat_0(2) - proj.CenterLambda
  Product : Product
  Projection : MATLAB Function  TreatAsAtomicUnit=on
  Scope : Scope
  Sum : Sum
  Sum1 : Sum  Inputs=|+-
  Sum2 : Sum  Inputs=+-
  lambda2_proj : Outport
  wires:
  Integrator/1 -> Sum2/1, Sum/2
  Constant/1 -> Sum2/2, Sum/1
  Gain/1 -> Sum1/2
  lambda2/1 -> Sum1/1
  Sum1/1 -> Projection/2(y)
  [ep_mag] -> Product/2
  Product/1 -> Gain/1
  Sum2/1 -> Product/1
  Sum/1 -> lambda2_proj/1, Scope/1, Projection/1(theta)
  Projection/1(y_proj) -> Integrator/1

== system RB_dyn/Predictor/Adaptive Laws/Projection and integration /Projection lambda3 ==
  lambda3 : Inport
  Constant : Constant  Value=proj.CenterLambda
  Gain : Gain  Gain=proj.sigma
  Integrator : Integrator  InitialCondition=LAMBDA_hat_0(3) - proj.CenterLambda
  Product : Product
  Projection : MATLAB Function  TreatAsAtomicUnit=on
  Sum : Sum
  Sum2 : Sum  Inputs=+-
  Sum3 : Sum  Inputs=|+-
  lambda3_proj : Outport
  wires:
  Integrator/1 -> Sum2/1, Sum/2
  Constant/1 -> Sum2/2, Sum/1
  Gain/1 -> Sum3/2
  Sum3/1 -> Projection/2(y)
  lambda3/1 -> Sum3/1
  [ep_mag] -> Product/2
  Product/1 -> Gain/1
  Sum2/1 -> Product/1
  Sum/1 -> lambda3_proj/1, Projection/1(theta)
  Projection/1(y_proj) -> Integrator/1

== system RB_dyn/Predictor/Adaptive Laws/Projection and integration 1/Projection Cx ==
  theta_cx : Inport
  Constant : Constant  Value=proj.CenterCxy
  Gain : Gain  Gain=proj.sigma
  Integrator : Integrator  InitialCondition=Theta_0(1) - proj.CenterCxy
  Product : Product
  Projection : MATLAB Function  TreatAsAtomicUnit=on
  Sum : Sum
  Sum1 : Sum  Inputs=|+-
  Sum2 : Sum  Inputs=|+-
  theta_cx_proj : Outport
  wires:
  Projection/1(y_proj) -> Integrator/1
  Integrator/1 -> Sum2/1, Sum/2
  Constant/1 -> Sum2/2, Sum/1
  Sum/1 -> theta_cx_proj/1, Projection/1(theta)
  theta_cx/1 -> Sum1/1
  Sum1/1 -> Projection/2(y)
  [ep_mag] -> Product/2
  Sum2/1 -> Product/1
  Product/1 -> Gain/1
  Gain/1 -> Sum1/2

== system RB_dyn/Predictor/Adaptive Laws/Projection and integration 1/Projection Cy ==
  theta_cy : Inport
  Constant : Constant  Value=proj.CenterCxy
  Gain : Gain  Gain=proj.sigma
  Integrator : Integrator  InitialCondition=Theta_0(2) - proj.CenterCxy
  Product : Product
  Projection : MATLAB Function  TreatAsAtomicUnit=on
  Sum : Sum
  Sum1 : Sum  Inputs=|+-
  Sum2 : Sum  Inputs=|+-
  theta_cy_proj : Outport
  wires:
  Projection/1(y_proj) -> Integrator/1
  Sum/1 -> theta_cy_proj/1, Projection/1(theta)
  Gain/1 -> Sum1/2
  Constant/1 -> Sum2/2, Sum/1
  Sum2/1 -> Product/1
  Integrator/1 -> Sum2/1, Sum/2
  [ep_mag] -> Product/2
  Product/1 -> Gain/1
  theta_cy/1 -> Sum1/1
  Sum1/1 -> Projection/2(y)

== system RB_dyn/Predictor/Adaptive Laws/Projection and integration 1/Projection Cz ==
  Cz : Inport
  Gain : Gain  Gain=GAMMA_a(6,6)
  Integrator : Integrator  InitialCondition=Theta_0(3)
  Cz_out : Outport
  wires:
  Cz/1 -> Gain/1
  Integrator/1 -> Cz_out/1
  Gain/1 -> Integrator/1

== system RB_dyn/Predictor/Adaptive Laws/Projection and integration 1/Projection Dx ==
  Dx : Inport
  Constant : Constant  Value=proj.CenterDxy
  Gain : Gain  Gain=proj.sigma
  Integrator : Integrator  InitialCondition=Theta_0(4) - proj.CenterDxy
  Product : Product
  Projection : MATLAB Function  TreatAsAtomicUnit=on
  Sum : Sum
  Sum1 : Sum  Inputs=|+-
  Sum2 : Sum  Inputs=|+-
  Dx_proj : Outport
  wires:
  Projection/1(y_proj) -> Integrator/1
  Sum/1 -> Dx_proj/1, Projection/1(theta)
  Gain/1 -> Sum1/2
  Constant/1 -> Sum2/2, Sum/1
  Sum2/1 -> Product/1
  Integrator/1 -> Sum2/1, Sum/2
  [ep_mag] -> Product/2
  Product/1 -> Gain/1
  Dx/1 -> Sum1/1
  Sum1/1 -> Projection/2(y)

== system RB_dyn/Predictor/Adaptive Laws/Projection and integration 1/Projection Dy ==
  Dy : Inport
  Constant : Constant  Value=proj.CenterDxy
  Gain : Gain  Gain=proj.sigma
  Integrator : Integrator  InitialCondition=Theta_0(5) - proj.CenterDxy
  Product : Product
  Projection : MATLAB Function  TreatAsAtomicUnit=on
  Sum : Sum
  Sum1 : Sum  Inputs=|+-
  Sum2 : Sum  Inputs=|+-
  Dy_proj : Outport
  wires:
  Projection/1(y_proj) -> Integrator/1
  Sum/1 -> Dy_proj/1, Projection/1(theta)
  Gain/1 -> Sum1/2
  Constant/1 -> Sum2/2, Sum/1
  Sum2/1 -> Product/1
  Integrator/1 -> Sum2/1, Sum/2
  [ep_mag] -> Product/2
  Product/1 -> Gain/1
  Dy/1 -> Sum1/1
  Sum1/1 -> Projection/2(y)

== system RB_dyn/Predictor/Adaptive Laws/Projection and integration 1/Projection Dz ==
  Dz : Inport
  Constant : Constant  Value=proj.CenterDz
  Gain : Gain  Gain=proj.sigma
  Integrator : Integrator  InitialCondition=Theta_0(6) - proj.CenterDz
  Product : Product
  Projection : MATLAB Function  TreatAsAtomicUnit=on
  Sum : Sum
  Sum1 : Sum  Inputs=|+-
  Sum2 : Sum  Inputs=|+-
  Dz_proj : Outport
  wires:
  Projection/1(y_proj) -> Integrator/1
  Sum/1 -> Dz_proj/1, Projection/1(theta)
  Gain/1 -> Sum1/2
  Constant/1 -> Sum2/2, Sum/1
  Sum2/1 -> Product/1
  Integrator/1 -> Sum2/1, Sum/2
  [ep_mag] -> Product/2
  Product/1 -> Gain/1
  Dz/1 -> Sum1/1
  Sum1/1 -> Projection/2(y)

== system RB_dyn/Predictor/Adaptive Laws/Projection and integration 1/Projection lambda1 ==
  lambda1 : Inport
  Constant : Constant  Value=proj.CenterLambda
  Gain : Gain  Gain=proj.sigma
  Integrator : Integrator  InitialCondition=LAMBDA_hat_0(1) - proj.CenterLambda
  Product : Product
  Projection : MATLAB Function  TreatAsAtomicUnit=on
  Sum : Sum
  Sum1 : Sum  Inputs=+-
  Sum2 : Sum  Inputs=+-
  lambda1_proj : Outport
  wires:
  lambda1/1 -> Sum1/1
  Integrator/1 -> Sum2/1, Sum/2
  Constant/1 -> Sum2/2, Sum/1
  Sum/1 -> lambda1_proj/1, Projection/1(theta)
  Projection/1(y_proj) -> Integrator/1
  Gain/1 -> Sum1/2
  Sum1/1 -> Projection/2(y)
  Sum2/1 -> Product/1
  Product/1 -> Gain/1
  [ep_mag] -> Product/2

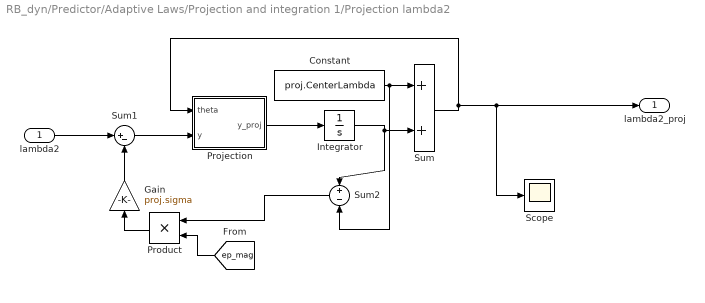
== system RB_dyn/Predictor/Adaptive Laws/Projection and integration 1/Projection lambda2 ==
  lambda2 : Inport
  Constant : Constant  Value=proj.CenterLambda
  Gain : Gain  Gain=proj.sigma
  Integrator : Integrator  InitialCondition=LAMBDA_hat_0(2) - proj.CenterLambda
  Product : Product
  Projection : MATLAB Function  TreatAsAtomicUnit=on
  Scope : Scope
  Sum : Sum
  Sum1 : Sum  Inputs=|+-
  Sum2 : Sum  Inputs=+-
  lambda2_proj : Outport
  wires:
  Integrator/1 -> Sum2/1, Sum/2
  Constant/1 -> Sum2/2, Sum/1
  Sum/1 -> Scope/1, lambda2_proj/1, Projection/1(theta)
  Projection/1(y_proj) -> Integrator/1
  Gain/1 -> Sum1/2
  lambda2/1 -> Sum1/1
  Sum1/1 -> Projection/2(y)
  [ep_mag] -> Product/2
  Sum2/1 -> Product/1
  Product/1 -> Gain/1

== system RB_dyn/Predictor/Adaptive Laws/Projection and integration 1/Projection lambda3 ==
  lambda3 : Inport
  Constant : Constant  Value=proj.CenterLambda
  Gain : Gain  Gain=proj.sigma
  Integrator : Integrator  InitialCondition=LAMBDA_hat_0(3) - proj.CenterLambda
  Product : Product
  Projection : MATLAB Function  TreatAsAtomicUnit=on
  Sum : Sum
  Sum2 : Sum  Inputs=+-
  Sum3 : Sum  Inputs=|+-
  lambda3_proj : Outport
  wires:
  Integrator/1 -> Sum2/1, Sum/2
  Constant/1 -> Sum2/2, Sum/1
  Sum/1 -> lambda3_proj/1, Projection/1(theta)
  Projection/1(y_proj) -> Integrator/1
  Gain/1 -> Sum3/2
  Sum3/1 -> Projection/2(y)
  lambda3/1 -> Sum3/1
  [ep_mag] -> Product/2
  Sum2/1 -> Product/1
  Product/1 -> Gain/1

== matlab function RB_dyn/Allocation + Actuator Dynamics/Allocation/MATLAB Function ==
  data: T input; Omega output
function Omega = T_Omega(T)
k_f = 3.65e-6; 
% 2. BLINDAJE TOTAL (Aquí está la magia)
    % Paso A: Eliminar cualquier parte imaginaria residual (si la hubiera)
    T_real = real(T);
    T_safe = max(T_real, 0);

    
    % 3. CÁLCULO
    Omega = sqrt(T_safe / k_f);

== matlab function RB_dyn/Dinámica UAV/Rigid Body dynamics&kinematics /MATLAB Function1 ==
  data: omega input; quat input; q_dot output
 function q_dot = quat_kin(omega, quat)
%#codegen

eta = quat(1);
e= quat(2:4);

W=[-e';
   skew(e) + eta*eye(3)];
% W = [-e(1), -e(2), -e(3);
%       eta,  -e(3),  e(2);
%       e(3),  eta,  -e(1);
%      -e(2),  e(1),   eta];

q_dot = 0.5*W*omega;

end

function S=skew(s)
S=[0  -s(3)  s(2);
    s(3)   0 -s(1);
    -s(2)  s(1)  0];
end

== matlab function RB_dyn/Atittude Planner & Controller/Atittude Controller/Original error1 ==
  data: E output; Rd input; R input
function E = error(Rd, R)

S = 1/2*(transpose(Rd)*R - transpose(R)*Rd);
E = [S(3, 2);S(1, 3);S(2, 1)];

end

== matlab function RB_dyn/Predictor/Diag1 ==
  data: u input; y output
function y = fcn(u)

y = diag(u);

== matlab function RB_dyn/Position Controller/Pos Controller/MATLAB Function2 ==
  data: u input; y output
function y = fcn(u)
y = norm(u);

== matlab function RB_dyn/Evalutaion/MATLAB Function2 ==
  data: p_real input; coste output; p_ref input; t input; e output
function [coste, e] = fcn(p_real, p_ref, t)
    

    e = p_real - p_ref; % [ex; ey; ez]
    coste = norm(e)^2;

== matlab function RB_dyn/Predictor/Phi_p ==
  data: v input size=[3,1]; phi output
function phi = fcn(v)

phi = [1 0 0 -v(1) zeros(1,2); 0 1 zeros(1,2) -v(2) 0;0 0 -1 zeros(1,2) -v(3)]';

== matlab function RB_dyn/V limitation/V_limitation ==
  data: v_cmd0 input; v_cmd output; Vmax parameter
function v_cmd = fcn(v_cmd0, Vmax)

v_cmd0_norm = v_cmd0/(norm(v_cmd0) + 1e-6);
v_cmd_norm = Vmax*tanh(norm(v_cmd0)/Vmax);
v_cmd = v_cmd0_norm*v_cmd_norm;

== matlab function RB_dyn/Predictor/Adaptive Laws/Projection and integration /Projection lambda1/Projection ==
  data: theta input; y_proj output; y input; GAMMA_a parameter; proj parameter
function y_proj = proj(theta,y,GAMMA_a, proj)
Gamma = GAMMA_a(1,1);
eps_proj = proj.eps;
theta_M = proj.RLambda;
center = proj.CenterLambda;
theta = theta - center;

f = 1/(eps_proj*theta_M^2)*((1+eps_proj)*(theta')*theta-theta_M^2);
grad_f = 2/(eps_proj*theta_M^2)*(1+eps_proj)*theta;

if f>0 && y'*Gamma*grad_f>0
    y_proj = Gamma*y - f*Gamma*(grad_f)*grad_f'/(grad_f'*Gamma*grad_f)*Gamma*y;
else
    y_proj = Gamma*y;
  
end

== matlab function RB_dyn/Predictor/Adaptive Laws/Projection and integration /Projection lambda2/Projection ==
  data: theta input; y_proj output; y input; GAMMA_a parameter; proj parameter
function y_proj = proj(theta,y,GAMMA_a, proj)
Gamma = GAMMA_a(2,2);
eps_proj = proj.eps;
theta_M = proj.RLambda;
center = proj.CenterLambda;
theta = theta - center;

f = 1/(eps_proj*theta_M^2)*((1+eps_proj)*(theta')*theta-theta_M^2);
grad_f = 2/(eps_proj*theta_M^2)*(1+eps_proj)*theta;

if f>0 && y'*Gamma*grad_f>0
    y_proj = Gamma*y - f*Gamma*(grad_f)*grad_f'/(grad_f'*Gamma*grad_f)*Gamma*y;
else
    y_proj = Gamma*y;
  
end

== matlab function RB_dyn/Predictor/Adaptive Laws/Projection and integration /Projection lambda3/Projection ==
  data: theta input; y_proj output; y input; GAMMA_a parameter; proj parameter
function y_proj = proj(theta,y,GAMMA_a, proj)
Gamma = GAMMA_a(3,3);
eps_proj = proj.eps;
theta_M = proj.RLambda;
center = proj.CenterLambda;
theta = theta - center;

f = 1/(eps_proj*theta_M^2)*((1+eps_proj)*(theta')*theta-theta_M^2);
grad_f = 2/(eps_proj*theta_M^2)*(1+eps_proj)*theta;

if f>0 && y'*Gamma*grad_f>0
    y_proj = Gamma*y - f*Gamma*(grad_f)*grad_f'/(grad_f'*Gamma*grad_f)*Gamma*y;
else
    y_proj = Gamma*y;
  
end

== matlab function RB_dyn/Predictor/Adaptive Laws/Projection and integration /Projection Cx/Projection ==
  data: theta input; y_proj output; y input; GAMMA_a parameter; proj parameter
function y_proj = proj(theta,y,GAMMA_a, proj)
Gamma = GAMMA_a(4,4);
eps_proj = proj.eps;
theta_M = proj.RCxy;
center = proj.CenterCxy;
theta = theta - center;

f = 1/(eps_proj*theta_M^2)*((1+eps_proj)*(theta')*theta-theta_M^2);
grad_f = 2/(eps_proj*theta_M^2)*(1+eps_proj)*theta;

if f>0 && y'*Gamma*grad_f>0
    y_proj = Gamma*y - f*Gamma*(grad_f)*grad_f'/(grad_f'*Gamma*grad_f)*Gamma*y;
else
    y_proj = Gamma*y;
  
end

== matlab function RB_dyn/Dinámica UAV/Rigid Body dynamics&kinematics /MATLAB Function ==
  data: quat input; euler output
function euler = quatToEuler( quat )
%	Converts a quaternion vector to ZYX Euler angles (RPY)

euler = quat2eul(quat','XYZ');

end

== matlab function RB_dyn/Predictor/Adaptive Laws/Projection and integration /Projection Cy/Projection ==
  data: theta input; y_proj output; y input; GAMMA_a parameter; proj parameter
function y_proj = proj(theta,y,GAMMA_a, proj)
Gamma = GAMMA_a(5,5);
eps_proj = proj.eps;
theta_M = proj.RCxy;
center = proj.CenterCxy;
theta = theta - center;

f = 1/(eps_proj*theta_M^2)*((1+eps_proj)*(theta')*theta-theta_M^2);
grad_f = 2/(eps_proj*theta_M^2)*(1+eps_proj)*theta;

if f>0 && y'*Gamma*grad_f>0
    y_proj = Gamma*y - f*Gamma*(grad_f)*grad_f'/(grad_f'*Gamma*grad_f)*Gamma*y;
else
    y_proj = Gamma*y;
  
end

== matlab function RB_dyn/Predictor/Adaptive Laws/Projection and integration /Projection Dx/Projection ==
  data: theta input; y_proj output; y input; GAMMA_a parameter; proj parameter
function y_proj = proj(theta,y,GAMMA_a, proj)
Gamma = GAMMA_a(7,7);
eps_proj = proj.eps;
theta_M = proj.RDxy;
center = proj.CenterDxy;
theta = theta - center;

f = 1/(eps_proj*theta_M^2)*((1+eps_proj)*(theta')*theta-theta_M^2);
grad_f = 2/(eps_proj*theta_M^2)*(1+eps_proj)*theta;

if f>0 && y'*Gamma*grad_f>0
    y_proj = Gamma*y - f*Gamma*(grad_f)*grad_f'/(grad_f'*Gamma*grad_f)*Gamma*y;
else
    y_proj = Gamma*y;
  
end

== matlab function RB_dyn/Predictor/Adaptive Laws/Projection and integration /Projection Dy/Projection ==
  data: theta input; y_proj output; y input; GAMMA_a parameter; proj parameter
function y_proj = proj(theta,y,GAMMA_a, proj)
Gamma = GAMMA_a(8,8);
eps_proj = proj.eps;
theta_M = proj.RDxy;
center = proj.CenterDxy;
theta = theta - center;

f = 1/(eps_proj*theta_M^2)*((1+eps_proj)*(theta')*theta-theta_M^2);
grad_f = 2/(eps_proj*theta_M^2)*(1+eps_proj)*theta;

if f>0 && y'*Gamma*grad_f>0
    y_proj = Gamma*y - f*Gamma*(grad_f)*grad_f'/(grad_f'*Gamma*grad_f)*Gamma*y;
else
    y_proj = Gamma*y;
  
end

== matlab function RB_dyn/Predictor/Adaptive Laws/Projection and integration /Projection Dz/Projection ==
  data: theta input; y_proj output; y input; GAMMA_a parameter; proj parameter
function y_proj = proj(theta,y,GAMMA_a, proj)
Gamma = GAMMA_a(9,9);
eps_proj = proj.eps;
theta_M = proj.RDz;
center = proj.CenterDz;
theta = theta - center;

f = 1/(eps_proj*theta_M^2)*((1+eps_proj)*(theta')*theta-theta_M^2);
grad_f = 2/(eps_proj*theta_M^2)*(1+eps_proj)*theta;

if f>0 && y'*Gamma*grad_f>0
    y_proj = Gamma*y - f*Gamma*(grad_f)*grad_f'/(grad_f'*Gamma*grad_f)*Gamma*y;
else
    y_proj = Gamma*y;
  
end

== matlab function RB_dyn/Predictor/Adaptive Laws/MATLAB Function ==
  data: u input; y output
function y = fcn(u)

y = norm(u);

== matlab function RB_dyn/Predictor/Adaptive Laws/Projection and integration 1/Projection Cx/Projection ==
  data: theta input; y_proj output; y input; GAMMA_a parameter; proj parameter
function y_proj = proj(theta,y,GAMMA_a, proj)
Gamma = GAMMA_a(4,4);
eps_proj = proj.eps;
theta_M = proj.RCxy;
center = proj.CenterCxy;
theta = theta - center;

f = 1/(eps_proj*theta_M^2)*((1+eps_proj)*(theta')*theta-theta_M^2);
grad_f = 2/(eps_proj*theta_M^2)*(1+eps_proj)*theta;

if f>0 && y'*Gamma*grad_f>0
    y_proj = Gamma*y - f*Gamma*(grad_f)*grad_f'/(grad_f'*Gamma*grad_f)*Gamma*y;
else
    y_proj = Gamma*y;
  
end

== matlab function RB_dyn/Predictor/Adaptive Laws/Projection and integration 1/Projection Cy/Projection ==
  data: theta input; y_proj output; y input; GAMMA_a parameter; proj parameter
function y_proj = proj(theta,y,GAMMA_a, proj)
Gamma = GAMMA_a(5,5);
eps_proj = proj.eps;
theta_M = proj.RCxy;
center = proj.CenterCxy;
theta = theta - center;

f = 1/(eps_proj*theta_M^2)*((1+eps_proj)*(theta')*theta-theta_M^2);
grad_f = 2/(eps_proj*theta_M^2)*(1+eps_proj)*theta;

if f>0 && y'*Gamma*grad_f>0
    y_proj = Gamma*y - f*Gamma*(grad_f)*grad_f'/(grad_f'*Gamma*grad_f)*Gamma*y;
else
    y_proj = Gamma*y;
  
end

== matlab function RB_dyn/Dinámica UAV/Rigid Body dynamics&kinematics /MATLAB Function2 ==
  data: q input; q_norm output
function q_norm = quat_norm( q )

norm = sqrt( q(1)^2 + q(2)^2 + q(3)^2 + q(4)^2 );

q_norm = 1/norm * q;

== matlab function RB_dyn/Predictor/Adaptive Laws/Projection and integration 1/Projection Dx/Projection ==
  data: theta input; y_proj output; y input; GAMMA_a parameter; proj parameter
function y_proj = proj(theta,y,GAMMA_a, proj)
Gamma = GAMMA_a(7,7);
eps_proj = proj.eps;
theta_M = proj.RDxy;
center = proj.CenterDxy;
theta = theta - center;

f = 1/(eps_proj*theta_M^2)*((1+eps_proj)*(theta')*theta-theta_M^2);
grad_f = 2/(eps_proj*theta_M^2)*(1+eps_proj)*theta;

if f>0 && y'*Gamma*grad_f>0
    y_proj = Gamma*y - f*Gamma*(grad_f)*grad_f'/(grad_f'*Gamma*grad_f)*Gamma*y;
else
    y_proj = Gamma*y;
  
end

== matlab function RB_dyn/Predictor/Adaptive Laws/Projection and integration 1/Projection Dy/Projection ==
  data: theta input; y_proj output; y input; GAMMA_a parameter; proj parameter
function y_proj = proj(theta,y,GAMMA_a, proj)
Gamma = GAMMA_a(8,8);
eps_proj = proj.eps;
theta_M = proj.RDxy;
center = proj.CenterDxy;
theta = theta - center;

f = 1/(eps_proj*theta_M^2)*((1+eps_proj)*(theta')*theta-theta_M^2);
grad_f = 2/(eps_proj*theta_M^2)*(1+eps_proj)*theta;

if f>0 && y'*Gamma*grad_f>0
    y_proj = Gamma*y - f*Gamma*(grad_f)*grad_f'/(grad_f'*Gamma*grad_f)*Gamma*y;
else
    y_proj = Gamma*y;
  
end
